simulink library "mec_pointmass_generic_ATvoith_DIWA_NXT"  (R2016a)
settings: Solver=ode45  SolverMode=SingleTasking  StartTime=0.0  StopTime=10.0  RelTol=1e-3
undefined symbols (not defined in the file): sMP
(part 4 of 4)

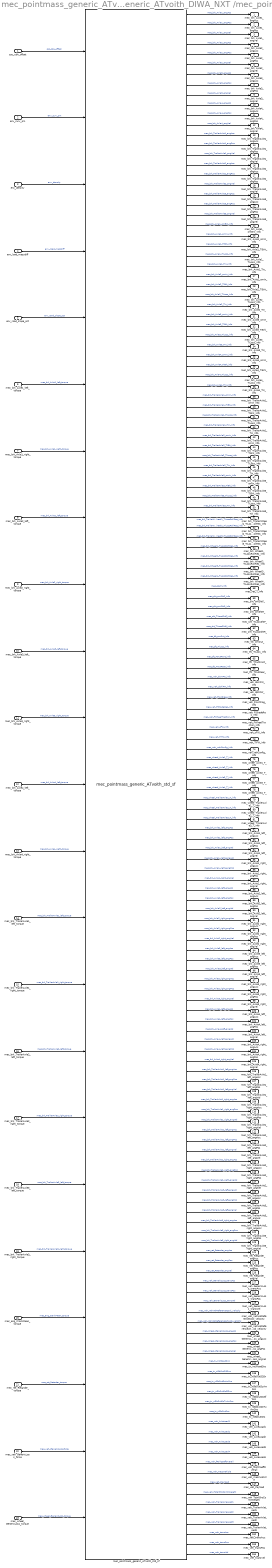
== system mec_pointmass_generic_ATvoith_DIWA_NXT/mec_pointmass_generic_ATvoith_DIWA_NXT /mec_pointmass_generic_ATvoith_std ==
  cpc_cdA_offset : Inport
  env_curv_pm : Inport  Port=2
  env_density : Inport  Port=3
  env_load_massdiff : Inport  Port=4
  env_road_slope_pct : Inport  Port=5
  mec_brk_Axle1_left_torque : Inport  Port=6
  mec_brk_Axle1_right_torque : Inport  Port=7
  mec_brk_Axle2_left_torque : Inport  Port=8
  mec_brk_Axle2_right_torque : Inport  Port=9
  mec_brk_Axle3_left_torque : Inport  Port=10
  mec_brk_Axle3_right_torque : Inport  Port=11
  mec_brk_Axle4_left_torque : Inport  Port=12
  mec_brk_Axle4_right_torque : Inport  Port=13
  mec_brk_TrailerAxle1_left_torque : Inport  Port=14
  mec_brk_TrailerAxle1_right_torque : Inport  Port=15
  mec_brk_TrailerAxle2_left_torque : Inport  Port=16
  mec_brk_TrailerAxle2_right_torque : Inport  Port=17
  mec_brk_TrailerAxle3_left_torque : Inport  Port=18
  mec_brk_TrailerAxle3_right_torque : Inport  Port=19
  mec_eng_CrankMean_torque : Inport  Port=20
  mec_ret_Retarder_torque : Inport  Port=21
  mec_veh_GenericLoss_force : Inport  Port=22
  mec_wheel_GenericLoss_torque : Inport  Port=23
  mec_pointmass_generic_ATvoith_std_sf : S-Function  FunctionName=mec_pointmass_generic_ATvoith_std_sf  Parameters=s1 s2 p1 p2 p3 p4 p5 p6 p7 p8 p9 p10 p11 p12 p13 p14 p15 p16 p17 p18 p19 p20 p21 p22 p23 p24 p25 p26 p27 p28 p29 p30 p31 p32 p33 p34 p35 p36 p37 p38 p39 p40 p41 p42 p43 p44 p45 p46 p47 p48 p49 p50 p51 p52 p53 p54 p55 p56 p57 p58 p59 p60 p61 p62 p63 p64 p65 p66 p67 p68 p69 p70 p71 p72 p73 p74 p75 p76 p77 p78 p79 p80 p81 p82 p83 p84 p85 p86 p87 p88 p89 p90 p91 p92 p93 p94 p95 p96 p97 p98 p99 p100 p101 p102 p103 p104 p105 p106 p107 p108 p109 p110 p111 p112 p113 p114 p115 p116 p117 p118 p119 p120 p121 p122 p123 p124 p125 p126 p127 p128 p129 p130 p131 p132 p133 p134 p135 p136 p137 p138 p139 p140 p141 p142 p143 p144 p145 p146 p147 p148 p149 p150 p151 p152 p153 p154 p155 p156 p157 p158 p159 p160 p161 p162 p163 p164 p165 p166 p167 p168 p169 p170 p171 p172 p173 p174 p175 p176 p177 p178 p179 p180 p181 p182 p183 p184 p185 p186 p187 p188 p189 p190 p191 p192 p193 p194 p195 p196 p197 p198 p199 p200 p201 p202 p203 p204 p205 p206 p207 p208 p209 p210 p211 p212 p213 p214 p215 p216 p217 p218 p219 p220 p221 p222 p223 p224 p225 p226 p227 p228 p229 p230 p231 p232 p233 p234 p235 p236 p237 p238 p239 p240 p241 p242 p243 p244 p245 p246 p247 p248 p249 p250 p251 p252 p253 p254 p255 p256 p257 p258 p259 p260 p261 p262 p263 p264 p265 p266 p267 p268 p269 p270 p271 p272 p273 p274 p275 p276 p277 p278 p279 p280 p281 p282 p283 p284 p285 p286 p287 p288 p289 p290 p291 p292 p293 p294 p295 p296 p297 p298 p299 p300  SFunctionModules=<binary blob, 819 chars, not shown>  SFunctionDeploymentMode=off  EnableBusSupport=off  mask{s1=s1, s2=s2, initCmd='Parameters_mec_pointmass_generic_ATvoith_std_sf', p1=p1, p2=p2, p3=p3, p4=p4, p5=p5, p6=p6, p7=p7, p8=p8, p9=p9, p10=p10, p11=p11, p12=p12, p13=p13, p14=p14, p15=p15, p16=p16, p17=p17, p18=p18, p19=p19, p20=p20, p21=p21, p22=p22, p23=p23, p24=p24, p25=p25, p26=p26, p27=p27, p28=p28, p29=p29, p30=p30, p31=p31, p32=p32, p33=p33, p34=p34, p35=p35, p36=p36, p37=p37, p38=p38, p39=p39, p40=p40, p41=p41, p42=p42, p43=p43, p44=p44, p45=p45, p46=p46, p47=p47, p48=p48, p49=p49, p50=p50, p51=p51, p52=p52, p53=p53, p54=p54, p55=p55, p56=p56, p57=p57, p58=p58, p59=p59, p60=p60, p61=p61, p62=p62, p63=p63, p64=p64, p65=p65, p66=p66, p67=p67, p68=p68, p69=p69, p70=p70, p71=p71, p72=p72, p73=p73, p74=p74, p75=p75, p76=p76, p77=p77, p78=p78, p79=p79, p80=p80, p81=p81, p82=p82, p83=p83, p84=p84, p85=p85, p86=p86, p87=p87, p88=p88, p89=p89, p90=p90, p91=p91, p92=p92, p93=p93, p94=p94, p95=p95, p96=p96, p97=p97, p98=p98, p99=p99, p100=p100, p101=p101, p102=p102, p103=p103, p104=p104, p105=p105, p106=p106, p107=p107, p108=p108, p109=p109, p110=p110, p111=p111, p112=p112, p113=p113, p114=p114, p115=p115, p116=p116, p117=p117, p118=p118, p119=p119, p120=p120, p121=p121, p122=p122, p123=p123, p124=p124, p125=p125, p126=p126, p127=p127, p128=p128, p129=p129, p130=p130, p131=p131, p132=p132, p133=p133, p134=p134, p135=p135, p136=p136, p137=p137, p138=p138, p139=p139, p140=p140, p141=p141, p142=p142, p143=p143, p144=p144, p145=p145, p146=p146, p147=p147, p148=p148, p149=p149, p150=p150, p151=p151, p152=p152, p153=p153, p154=p154, p155=p155, p156=p156, p157=p157, p158=p158, p159=p159, p160=p160, p161=p161, p162=p162, p163=p163, p164=p164, p165=p165, p166=p166, p167=p167, p168=p168, p169=p169, p170=p170, p171=p171, p172=p172, p173=p173, p174=p174, p175=p175, p176=p176, p177=p177, p178=p178, p179=p179, p180=p180, p181=p181, p182=p182, p183=p183, p184=p184, p185=p185, p186=p186, p187=p187, p188=p188, p189=p189, p190=p190, p191=p191, p192=p192, p193=p193, p194=p194, p195=p195, p196=p196, p197=p197, p198=p198, p199=p199, p200=p200, p201=p201, p202=p202, p203=p203, p204=p204, p205=p205, p206=p206, p207=p207, p208=p208, p209=p209, p210=p210, p211=p211, p212=p212, p213=p213, p214=p214, p215=p215, p216=p216, p217=p217, p218=p218, p219=p219, p220=p220, p221=p221, p222=p222, p223=p223, p224=p224, p225=p225, p226=p226, p227=p227, p228=p228, p229=p229, p230=p230, p231=p231, p232=p232, p233=p233, p234=p234, p235=p235, p236=p236, p237=p237, p238=p238, p239=p239, p240=p240, p241=p241, p242=p242, p243=p243, p244=p244, p245=p245, p246=p246, p247=p247, p248=p248, p249=p249, p250=p250, p251=p251, p252=p252, p253=p253, p254=p254, p255=p255, p256=p256, p257=p257, p258=p258, p259=p259, p260=p260, p261=p261, p262=p262, p263=p263, p264=p264, p265=p265, p266=p266, p267=p267, p268=p268, p269=p269, p270=p270, p271=p271, p272=p272, p273=p273, p274=p274, p275=p275, p276=p276, p277=p277, p278=p278, p279=p279, p280=p280, p281=p281, p282=p282, p283=p283, p284=p284, p285=p285, p286=p286, p287=p287, p288=p288, p289=p289, p290=p290, p291=p291, p292=p292, p293=p293, p294=p294, p295=p295, p296=p296, p297=p297, p298=p298, p299=p299, p300=p300}
      mask prompts: s1 "Solver Type: settings_iMode [-]"; s2 "Solver Step Size: settings_dt [s]"; initCmd "Initialization command"; p1 "Ratio Differential Gear [-] export=true name=iDiff prio=1 dataSetName=axle_dummy dataClassType=axle dataClassName=$dataClassNameAxle$ moduleXmlReference=$moduleXmlReferenceAxle$ unit='-' description='Ratio Differential Gear': axle1.iDiff [-]"; p2 "Is driven Axle? [-] export=true name=isDriven prio=1 dataSetName=axle_dummy dataClassType=axle dataClassName=$dataClassNameAxle$ moduleXmlReference=$moduleXmlReferenceAxle$ unit='-' description='Is Driven Axle': axle1.isDriven [-]"; p3 "Is rear Axle? [-] export=true name=isRearAxle prio=1 dataSetName=axle_dummy dataClassType=axle dataClassName=$dataClassNameAxle$ moduleXmlReference=$moduleXmlReferenceAxle$ unit='-' description='Is Rear Axle': axle1.isRearAxle [-]"; p4 "Inertia Brake Disc  [kgm^2] export=true name=JBrakeDisc_kgm2 prio=1 dataSetName=brk_dummy dataClassType=brk dataClassName=$dataClassNameBrk$ moduleXmlReference=$moduleXmlReferenceBrk$ unit='kgm^2' description='Inertia Brake Disc': axle1.JBrakeDisc_kgm2 [kgm²]"; p5 "Inertia Hub  [kgm^2] export=true name=JHub_kgm2 prio=1 dataSetName=brk_dummy dataClassType=brk dataClassName=$dataClassNameBrk$ moduleXmlReference=$moduleXmlReferenceBrk$ unit='kgm^2' description='Inertia Hub': axle1.JHub_kgm2 [-]"; p6 "Inertia Side Shaft [kgm^2] export=true name=JSideShft_kgm2 prio=1 dataSetName=axle_dummy dataClassType=axle dataClassName=$dataClassNameAxle$ moduleXmlReference=$moduleXmlReferenceAxle$ unit='kgm^2' description='Inertia Side Shaft': axle1.JSideShft_kgm2 [kgm²]"; p7 "Ratio Differential Gear [-] export=true name=iDiff prio=1 dataSetName=axle_dummy dataClassType=axle dataClassName=$dataClassNameAxle$ moduleXmlReference=$moduleXmlReferenceAxle$ unit='-' description='Ratio Differential Gear': axle2.iDiff [-]"; p8 "Is driven Axle? [-] export=true name=isDriven prio=1 dataSetName=axle_dummy dataClassType=axle dataClassName=$dataClassNameAxle$ moduleXmlReference=$moduleXmlReferenceAxle$ unit='-' description='Is Driven Axle': axle2.isDriven [-]"; p9 "Is rear Axle? [-] export=true name=isRearAxle prio=1 dataSetName=axle_dummy dataClassType=axle dataClassName=$dataClassNameAxle$ moduleXmlReference=$moduleXmlReferenceAxle$ unit='-' description='Is Rear Axle': axle2.isRearAxle [-]"; p10 "Inertia Brake Disc  [kgm^2] export=true name=JBrakeDisc_kgm2 prio=1 dataSetName=brk_dummy dataClassType=brk dataClassName=$dataClassNameBrk$ moduleXmlReference=$moduleXmlReferenceBrk$ unit='kgm^2' description='Inertia Brake Disc': axle2.JBrakeDisc_kgm2 [kgm²]"; p11 "Inertia Hub  [kgm^2] export=true name=JHub_kgm2 prio=1 dataSetName=brk_dummy dataClassType=brk dataClassName=$dataClassNameBrk$ moduleXmlReference=$moduleXmlReferenceBrk$ unit='kgm^2' description='Inertia Hub': axle2.JHub_kgm2 [-]"; p12 "Inertia Side Shaft [kgm^2] export=true name=JSideShft_kgm2 prio=1 dataSetName=axle_dummy dataClassType=axle dataClassName=$dataClassNameAxle$ moduleXmlReference=$moduleXmlReferenceAxle$ unit='kgm^2' description='Inertia Side Shaft': axle2.JSideShft_kgm2 [kgm²]"; p13 "Ratio Differential Gear [-] export=true name=iDiff prio=1 dataSetName=axle_dummy dataClassType=axle dataClassName=$dataClassNameAxle$ moduleXmlReference=$moduleXmlReferenceAxle$ unit='-' description='Ratio Differential Gear': axle3.iDiff [-]"; p14 "Is driven Axle? [-] export=true name=isDriven prio=1 dataSetName=axle_dummy dataClassType=axle dataClassName=$dataClassNameAxle$ moduleXmlReference=$moduleXmlReferenceAxle$ unit='-' description='Is Driven Axle': axle3.isDriven [-]"; p15 "Is rear Axle? [-] export=true name=isRearAxle prio=1 dataSetName=axle_dummy dataClassType=axle dataClassName=$dataClassNameAxle$ moduleXmlReference=$moduleXmlReferenceAxle$ unit='-' description='Is Rear Axle': axle3.isRearAxle [-]"; p16 "Inertia Brake Disc  [kgm^2] export=true name=JBrakeDisc_kgm2 prio=1 dataSetName=brk_dummy dataClassType=brk dataClassName=$dataClassNameBrk$ moduleXmlReference=$moduleXmlReferenceBrk$ unit='kgm^2' description='Inertia Brake Disc': axle3.JBrakeDisc_kgm2 [kgm²]"; p17 "Inertia Hub  [kgm^2] export=true name=JHub_kgm2 prio=1 dataSetName=brk_dummy dataClassType=brk dataClassName=$dataClassNameBrk$ moduleXmlReference=$moduleXmlReferenceBrk$ unit='kgm^2' description='Inertia Hub': axle3.JHub_kgm2 [-]"; p18 "Inertia Side Shaft [kgm^2] export=true name=JSideShft_kgm2 prio=1 dataSetName=axle_dummy dataClassType=axle dataClassName=$dataClassNameAxle$ moduleXmlReference=$moduleXmlReferenceAxle$ unit='kgm^2' description='Inertia Side Shaft': axle3.JSideShft_kgm2 [kgm²]"; p19 "Ratio Differential Gear [-] export=true name=iDiff prio=1 dataSetName=axle_dummy dataClassType=axle dataClassName=$dataClassNameAxle$ moduleXmlReference=$moduleXmlReferenceAxle$ unit='-' description='Ratio Differential Gear': axle4.iDiff [-]"; p20 "Is driven Axle? [-] export=true name=isDriven prio=1 dataSetName=axle_dummy dataClassType=axle dataClassName=$dataClassNameAxle$ moduleXmlReference=$moduleXmlReferenceAxle$ unit='-' description='Is Driven Axle': axle4.isDriven [-]"; p21 "Is rear Axle? [-] export=true name=isRearAxle prio=1 dataSetName=axle_dummy dataClassType=axle dataClassName=$dataClassNameAxle$ moduleXmlReference=$moduleXmlReferenceAxle$ unit='-' description='Is Rear Axle': axle4.isRearAxle [-]"; p22 "Inertia Brake Disc  [kgm^2] export=true name=JBrakeDisc_kgm2 prio=1 dataSetName=brk_dummy dataClassType=brk dataClassName=$dataClassNameBrk$ moduleXmlReference=$moduleXmlReferenceBrk$ unit='kgm^2' description='Inertia Brake Disc': axle4.JBrakeDisc_kgm2 [kgm²]"; p23 "Inertia Hub  [kgm^2] export=true name=JHub_kgm2 prio=1 dataSetName=brk_dummy dataClassType=brk dataClassName=$dataClassNameBrk$ moduleXmlReference=$moduleXmlReferenceBrk$ unit='kgm^2' description='Inertia Hub': axle4.JHub_kgm2 [-]"; p24 "Inertia Side Shaft [kgm^2] export=true name=JSideShft_kgm2 prio=1 dataSetName=axle_dummy dataClassType=axle dataClassName=$dataClassNameAxle$ moduleXmlReference=$moduleXmlReferenceAxle$ unit='kgm^2' description='Inertia Side Shaft': axle4.JSideShft_kgm2 [kgm²]"; p25 "Additive Controlable Air Resistance (init) export=$sw_cpc_cdA_offset$ name=cpc_cdA_offset prio=1 dataSetName=std dataClassType=initIO dataClassName=initIO unit='' description='Additive Controlable Air Resistance': interface_IO.cpc_cdA_offset_0 [-]"; p26 "Curve Curvature (init) export=$sw_env_curv_pm$ name=env_curv_pm prio=1 dataSetName=std dataClassType=initIO dataClassName=initIO unit='1/m' description='Curve Curvature': interface_IO.env_curv_pm_0 [-]"; p27 "Air density from environment (init) export=$sw_env_density$ name=env_density prio=1 dataSetName=std dataClassType=initIO dataClassName=initIO unit='kg/m^3' description='Air density from environment': interface_IO.env_density_0 [-]"; p28 "Mass Difference (init) export=$sw_env_load_massdiff$ name=env_load_massdiff prio=1 dataSetName=std dataClassType=initIO dataClassName=initIO unit='1/m' description='Curve Curvature': interface_IO.env_load_massdiff_0 [-]"; p29 "Slope of road from environment (init) export=$sw_env_road_slope_pct$ name=env_road_slope_pct prio=1 dataSetName=std dataClassType=initIO dataClassName=initIO unit='-' description='Slope of road from environment': interface_IO.env_road_slope_pct_0 [-]"; p30 "Acceleration Brake 1 (init) export=$sw_mec_brk_Axle1_angAcc$ name=mec_brk_Axle1_angAcc prio=1 dataSetName=std dataClassType=initIO dataClassName=initIO unit='rad/s^2' description='Acceleration Brake 1': interface_IO.mec_brk_Axle1_angAcc_0 [-]"; p31 "Angle Brake 1 (init) export=$sw_mec_brk_Axle1_angPos$ name=mec_brk_Axle1_angPos prio=1 dataSetName=std dataClassType=initIO dataClassName=initIO unit='rad' description='Angle Brake 1': interface_IO.mec_brk_Axle1_angPos_0 [-]"; p32 "Velocity Brake 1 (init) export=$sw_mec_brk_Axle1_angVel$ name=mec_brk_Axle1_angVel prio=1 dataSetName=std dataClassType=initIO dataClassName=initIO unit='rad/s' description='Velocity Brake 1': interface_IO.mec_brk_Axle1_angVel_0 [-]"; p33 "Acceleration Brake 1 left Wheel (init) export=$sw_mec_brk_Axle1_left_angAcc$ name=mec_brk_Axle1_left_angAcc prio=1 dataSetName=std dataClassType=initIO dataClassName=initIO unit='rad/s^2' description='Acceleration Brake 1 left Wheel': interface_IO.mec_brk_Axle1_left_angAcc_0 [-]"; p34 "Angle Brake 1 left Wheel (init) export=$sw_mec_brk_Axle1_left_angPos$ name=mec_brk_Axle1_left_angPos prio=1 dataSetName=std dataClassType=initIO dataClassName=initIO unit='rad' description='Angle Brake 1 left Wheel': interface_IO.mec_brk_Axle1_left_angPos_0 [-]"; p35 "Velocity Brake 1 left Wheel (init) export=$sw_mec_brk_Axle1_left_angVel$ name=mec_brk_Axle1_left_angVel prio=1 dataSetName=std dataClassType=initIO dataClassName=initIO unit='rad/s' description='Velocity Brake 1 left Wheel': interface_IO.mec_brk_Axle1_left_angVel_0 [-]"; p36 "Torque Brake 1 left Wheel (init) export=$sw_mec_brk_Axle1_left_torque$ name=mec_brk_Axle1_left_torque prio=1 dataSetName=std dataClassType=initIO dataClassName=initIO unit='Nm' description='Torque Brake 1 left Wheel': interface_IO.mec_brk_Axle1_left_torque_0 [-]"; p37 "Acceleration Brake 1 right Wheel (init) export=$sw_mec_brk_Axle1_right_angAcc$ name=mec_brk_Axle1_right_angAcc prio=1 dataSetName=std dataClassType=initIO dataClassName=initIO unit='rad/s^2' description='Acceleration Brake 1 right Wheel': interface_IO.mec_brk_Axle1_right_angAcc_0 [-]"; p38 "Angle Brake 1 right Wheel (init) export=$sw_mec_brk_Axle1_right_angPos$ name=mec_brk_Axle1_right_angPos prio=1 dataSetName=std dataClassType=initIO dataClassName=initIO unit='rad' description='Angle Brake 1 right Wheel': interface_IO.mec_brk_Axle1_right_angPos_0 [-]"; p39 "Velocity Brake 1 right Wheel (init) export=$sw_mec_brk_Axle1_right_angVel$ name=mec_brk_Axle1_right_angVel prio=1 dataSetName=std dataClassType=initIO dataClassName=initIO unit='rad/s' description='Velocity Brake 1 right Wheel': interface_IO.mec_brk_Axle1_right_angVel_0 [-]"; p40 "Torque Brake 1 left Wheel (init) export=$sw_mec_brk_Axle1_right_torque$ name=mec_brk_Axle1_right_torque prio=1 dataSetName=std dataClassType=initIO dataClassName=initIO unit='Nm' description='Torque Brake 1 left Wheel': interface_IO.mec_brk_Axle1_right_torque_0 [-]"; p41 "Acceleration Brake 2 (init) export=$sw_mec_brk_Axle2_angAcc$ name=mec_brk_Axle2_angAcc prio=1 dataSetName=std dataClassType=initIO dataClassName=initIO unit='rad/s^2' description='Acceleration Brake 2': interface_IO.mec_brk_Axle2_angAcc_0 [-]"; p42 "Angle Brake 2 (init) export=$sw_mec_brk_Axle2_angPos$ name=mec_brk_Axle2_angPos prio=1 dataSetName=std dataClassType=initIO dataClassName=initIO unit='rad' description='Angle Brake 2': interface_IO.mec_brk_Axle2_angPos_0 [-]"; p43 "Velocity Brake 2 (init) export=$sw_mec_brk_Axle2_angVel$ name=mec_brk_Axle2_angVel prio=1 dataSetName=std dataClassType=initIO dataClassName=initIO unit='rad/s' description='Velocity Brake 3': interface_IO.mec_brk_Axle2_angVel_0 [-]"; p44 "Acceleration Brake 2 left Wheel (init) export=$sw_mec_brk_Axle2_left_angAcc$ name=mec_brk_Axle2_left_angAcc prio=1 dataSetName=std dataClassType=initIO dataClassName=initIO unit='rad/s^2' description='Acceleration Brake 2 left Wheel': interface_IO.mec_brk_Axle2_left_angAcc_0 [-]"; p45 "Angle Brake 2 left Wheel (init) export=$sw_mec_brk_Axle2_left_angPos$ name=mec_brk_Axle2_left_angPos prio=1 dataSetName=std dataClassType=initIO dataClassName=initIO unit='rad' description='Angle Brake 2 left Wheel': interface_IO.mec_brk_Axle2_left_angPos_0 [-]"; p46 "Velocity Brake 2 left Wheel (init) export=$sw_mec_brk_Axle2_left_angVel$ name=mec_brk_Axle2_left_angVel prio=1 dataSetName=std dataClassType=initIO dataClassName=initIO unit='rad/s' description='Velocity Brake 3 left Wheel': interface_IO.mec_brk_Axle2_left_angVel_0 [-]"; p47 "Torque Brake 2 left Wheel (init) export=$sw_mec_brk_Axle2_left_torque$ name=mec_brk_Axle2_left_torque prio=1 dataSetName=std dataClassType=initIO dataClassName=initIO unit='Nm' description='Torque Brake 2 left Wheel': interface_IO.mec_brk_Axle2_left_torque_0 [-]"; p48 "Acceleration Brake 2 right Wheel (init) export=$sw_mec_brk_Axle2_right_angAcc$ name=mec_brk_Axle2_right_angAcc prio=1 dataSetName=std dataClassType=initIO dataClassName=initIO unit='rad/s^2' description='Acceleration Brake 2 right Wheel': interface_IO.mec_brk_Axle2_right_angAcc_0 [-]"; p49 "Angle Brake 2 right Wheel (init) export=$sw_mec_brk_Axle2_right_angPos$ name=mec_brk_Axle2_right_angPos prio=1 dataSetName=std dataClassType=initIO dataClassName=initIO unit='rad' description='Angle Brake 2 right Wheel': interface_IO.mec_brk_Axle2_right_angPos_0 [-]"; p50 "Velocity Brake 2 right Wheel (init) export=$sw_mec_brk_Axle2_right_angVel$ name=mec_brk_Axle2_right_angVel prio=1 dataSetName=std dataClassType=initIO dataClassName=initIO unit='rad/s' description='Velocity Brake 3 right Wheel': interface_IO.mec_brk_Axle2_right_angVel_0 [-]"; p51 "Torque Brake 2 right Wheel (init) export=$sw_mec_brk_Axle2_right_torque$ name=mec_brk_Axle2_right_torque prio=1 dataSetName=std dataClassType=initIO dataClassName=initIO unit='Nm' description='Torque Brake 2 right Wheel': interface_IO.mec_brk_Axle2_right_torque_0 [-]"; p52 "Acceleration Brake 3 (init) export=$sw_mec_brk_Axle3_angAcc$ name=mec_brk_Axle3_angAcc prio=1 dataSetName=std dataClassType=initIO dataClassName=initIO unit='rad/s^2' description='Acceleration Brake 3': interface_IO.mec_brk_Axle3_angAcc_0 [-]"; p53 "Angle Brake 3 (init) export=$sw_mec_brk_Axle3_angPos$ name=mec_brk_Axle3_angPos prio=1 dataSetName=std dataClassType=initIO dataClassName=initIO unit='rad' description='Angle Brake 3': interface_IO.mec_brk_Axle3_angPos_0 [-]"; p54 "Velocity Brake 3 (init) export=$sw_mec_brk_Axle3_angVel$ name=mec_brk_Axle3_angVel prio=1 dataSetName=std dataClassType=initIO dataClassName=initIO unit='rad/s' description='Velocity Brake 3': interface_IO.mec_brk_Axle3_angVel_0 [-]"; p55 "Acceleration Brake 3 left Wheel (init) export=$sw_mec_brk_Axle3_left_angAcc$ name=mec_brk_Axle3_left_angAcc prio=1 dataSetName=std dataClassType=initIO dataClassName=initIO unit='rad/s^2' description='Acceleration Brake 3 left Wheel': interface_IO.mec_brk_Axle3_left_angAcc_0 [-]"; p56 "Angle Brake 3 left Wheel (init) export=$sw_mec_brk_Axle3_left_angPos$ name=mec_brk_Axle3_left_angPos prio=1 dataSetName=std dataClassType=initIO dataClassName=initIO unit='rad' description='Angle Brake 3 left Wheel': interface_IO.mec_brk_Axle3_left_angPos_0 [-]"; p57 "Velocity Brake 3 left Wheel (init) export=$sw_mec_brk_Axle3_left_angVel$ name=mec_brk_Axle3_left_angVel prio=1 dataSetName=std dataClassType=initIO dataClassName=initIO unit='rad/s' description='Velocity Brake 3 left Wheel': interface_IO.mec_brk_Axle3_left_angVel_0 [-]"; p58 "Torque Brake 3 left Wheel (init) export=$sw_mec_brk_Axle3_left_torque$ name=mec_brk_Axle3_left_torque prio=1 dataSetName=std dataClassType=initIO dataClassName=initIO unit='Nm' description='Torque Brake 3 left Wheel': interface_IO.mec_brk_Axle3_left_torque_0 [-]"; p59 "Acceleration Brake 3 right Wheel (init) export=$sw_mec_brk_Axle3_right_angAcc$ name=mec_brk_Axle3_right_angAcc prio=1 dataSetName=std dataClassType=initIO dataClassName=initIO unit='rad/s^2' description='Acceleration Brake 3 right Wheel': interface_IO.mec_brk_Axle3_right_angAcc_0 [-]"; p60 "Angle Brake 3 right Wheel (init) export=$sw_mec_brk_Axle3_right_angPos$ name=mec_brk_Axle3_right_angPos prio=1 dataSetName=std dataClassType=initIO dataClassName=initIO unit='rad' description='Angle Brake 3 right Wheel': interface_IO.mec_brk_Axle3_right_angPos_0 [-]"; p61 "Velocity Brake 3 right Wheel (init) export=$sw_mec_brk_Axle3_right_angVel$ name=mec_brk_Axle3_right_angVel prio=1 dataSetName=std dataClassType=initIO dataClassName=initIO unit='rad/s' description='Velocity Brake 3 right Wheel': interface_IO.mec_brk_Axle3_right_angVel_0 [-]"; p62 "Torque Brake 3 right Wheel (init) export=$sw_mec_brk_Axle3_right_torque$ name=mec_brk_Axle3_right_torque prio=1 dataSetName=std dataClassType=initIO dataClassName=initIO unit='Nm' description='Torque Brake 3 right Wheel': interface_IO.mec_brk_Axle3_right_torque_0 [-]"; p63 "Acceleration Brake 4 (init) export=$sw_mec_brk_Axle4_angAcc$ name=mec_brk_Axle4_angAcc prio=1 dataSetName=std dataClassType=initIO dataClassName=initIO unit='rad/s^2' description='Acceleration Brake 4': interface_IO.mec_brk_Axle4_angAcc_0 [-]"; p64 "Angle Brake 4 (init) export=$sw_mec_brk_Axle4_angPos$ name=mec_brk_Axle4_angPos prio=1 dataSetName=std dataClassType=initIO dataClassName=initIO unit='rad' description='Angle Brake 4': interface_IO.mec_brk_Axle4_angPos_0 [-]"; p65 "Velocity Brake 4 (init) export=$sw_mec_brk_Axle4_angVel$ name=mec_brk_Axle4_angVel prio=1 dataSetName=std dataClassType=initIO dataClassName=initIO unit='rad/s' description='Velocity Brake 4': interface_IO.mec_brk_Axle4_angVel_0 [-]"; p66 "Acceleration Brake 4 left Wheel (init) export=$sw_mec_brk_Axle4_left_angAcc$ name=mec_brk_Axle4_left_angAcc prio=1 dataSetName=std dataClassType=initIO dataClassName=initIO unit='rad/s^2' description='Acceleration Brake 4 left Wheel': interface_IO.mec_brk_Axle4_left_angAcc_0 [-]"; p67 "Angle Brake 4 left Wheel (init) export=$sw_mec_brk_Axle4_left_angPos$ name=mec_brk_Axle4_left_angPos prio=1 dataSetName=std dataClassType=initIO dataClassName=initIO unit='rad' description='Angle Brake 4 left Wheel': interface_IO.mec_brk_Axle4_left_angPos_0 [-]"; p68 "Velocity Brake 4 left Wheel (init) export=$sw_mec_brk_Axle4_left_angVel$ name=mec_brk_Axle4_left_angVel prio=1 dataSetName=std dataClassType=initIO dataClassName=initIO unit='rad/s' description='Velocity Brake 4 left Wheel': interface_IO.mec_brk_Axle4_left_angVel_0 [-]"; p69 "Torque Brake 4 left Wheel (init) export=$sw_mec_brk_Axle4_left_torque$ name=mec_brk_Axle4_left_torque prio=1 dataSetName=std dataClassType=initIO dataClassName=initIO unit='Nm' description='Torque Brake 4 left Wheel': interface_IO.mec_brk_Axle4_left_torque_0 [-]"; p70 "Acceleration Brake 4 right Wheel (init) export=$sw_mec_brk_Axle4_right_angAcc$ name=mec_brk_Axle4_right_angAcc prio=1 dataSetName=std dataClassType=initIO dataClassName=initIO unit='rad/s^2' description='Acceleration Brake 4 right Wheel': interface_IO.mec_brk_Axle4_right_angAcc_0 [-]"; p71 "Angle Brake 4 right Wheel (init) export=$sw_mec_brk_Axle4_right_angPos$ name=mec_brk_Axle4_right_angPos prio=1 dataSetName=std dataClassType=initIO dataClassName=initIO unit='rad' description='Angle Brake 4 right Wheel': interface_IO.mec_brk_Axle4_right_angPos_0 [-]"; p72 "Velocity Brake 4 right Wheel (init) export=$sw_mec_brk_Axle4_right_angVel$ name=mec_brk_Axle4_right_angVel prio=1 dataSetName=std dataClassType=initIO dataClassName=initIO unit='rad/s' description='Velocity Brake 4 right Wheel': interface_IO.mec_brk_Axle4_right_angVel_0 [-]"; p73 "Torque Brake 4 right Wheel (init) export=$sw_mec_brk_Axle4_right_torque$ name=mec_brk_Axle4_right_torque prio=1 dataSetName=std dataClassType=initIO dataClassName=initIO unit='Nm' description='Torque Brake 4 right Wheel': interface_IO.mec_brk_Axle4_right_torque_0 [-]"; p74 "Acceleration Trailer Brake 1 (init) export=$sw_mec_brk_TrailerAxle1_angAcc$ name=mec_brk_TrailerAxle1_angAcc prio=1 dataSetName=std dataClassType=initIO dataClassName=initIO unit='rad/s^2' description='Acceleration Trailer Brake 1': interface_IO.mec_brk_TrailerAxle1_angAcc_0 [-]"; p75 "Angle Trailer Brake 1 (init) export=$sw_mec_brk_TrailerAxle1_angPos$ name=mec_brk_TrailerAxle1_angPos prio=1 dataSetName=std dataClassType=initIO dataClassName=initIO unit='rad' description='Angle Trailer Brake 1': interface_IO.mec_brk_TrailerAxle1_angPos_0 [-]"; p76 "Velocity Trailer Brake 1 (init) export=$sw_mec_brk_TrailerAxle1_angVel$ name=mec_brk_TrailerAxle1_angVel prio=1 dataSetName=std dataClassType=initIO dataClassName=initIO unit='rad/s' description='Velocity Trailer Brake 1': interface_IO.mec_brk_TrailerAxle1_angVel_0 [-]"; p77 "Acceleration Trailer Brake 1 left Wheel (init) export=$sw_mec_brk_TrailerAxle1_left_angAcc$ name=mec_brk_TrailerAxle1_left_angAcc prio=1 dataSetName=std dataClassType=initIO dataClassName=initIO unit='rad/s^2' description='Acceleration Trailer Brake 1 left Wheel': interface_IO.mec_brk_TrailerAxle1_left_angAcc_0 [-]"; p78 "Angle Trailer Brake 1 left Wheel (init) export=$sw_mec_brk_TrailerAxle1_left_angPos$ name=mec_brk_TrailerAxle1_left_angPos prio=1 dataSetName=std dataClassType=initIO dataClassName=initIO unit='rad' description='Angle Trailer Brake 1 left Wheel': interface_IO.mec_brk_TrailerAxle1_left_angPos_0 [-]"; p79 "Velocity Trailer Brake 1 left Wheel (init) export=$sw_mec_brk_TrailerAxle1_left_angVel$ name=mec_brk_TrailerAxle1_left_angVel prio=1 dataSetName=std dataClassType=initIO dataClassName=initIO unit='rad/s' description='Velocity Trailer Brake 1 left Wheel': interface_IO.mec_brk_TrailerAxle1_left_angVel_0 [-]"; p80 "Torque Trailer Brake 1 left Wheel (init) export=$sw_mec_brk_TrailerAxle1_left_torque$ name=mec_brk_TrailerAxle1_left_torque prio=1 dataSetName=std dataClassType=initIO dataClassName=initIO unit='Nm' description='Torque Trailer Brake 1 left Wheel': interface_IO.mec_brk_TrailerAxle1_left_torque_0 [-]"; p81 "Acceleration Trailer Brake 1 right Wheel (init) export=$sw_mec_brk_TrailerAxle1_right_angAcc$ name=mec_brk_TrailerAxle1_right_angAcc prio=1 dataSetName=std dataClassType=initIO dataClassName=initIO unit='rad/s^2' description='Acceleration Trailer Brake 1 right Wheel': interface_IO.mec_brk_TrailerAxle1_right_angAcc_0 [-]"; p82 "Angle Trailer Brake 1 right Wheel (init) export=$sw_mec_brk_TrailerAxle1_right_angPos$ name=mec_brk_TrailerAxle1_right_angPos prio=1 dataSetName=std dataClassType=initIO dataClassName=initIO unit='rad' description='Angle Trailer Brake 1 right Wheel': interface_IO.mec_brk_TrailerAxle1_right_angPos_0 [-]"; p83 "Velocity Trailer Brake 1 right Wheel (init) export=$sw_mec_brk_TrailerAxle1_right_angVel$ name=mec_brk_TrailerAxle1_right_angVel prio=1 dataSetName=std dataClassType=initIO dataClassName=initIO unit='rad/s' description='Velocity Trailer Brake 1 right Wheel': interface_IO.mec_brk_TrailerAxle1_right_angVel_0 [-]"; p84 "Torque Trailer Brake 1 right Wheel (init) export=$sw_mec_brk_TrailerAxle1_right_torque$ name=mec_brk_TrailerAxle1_right_torque prio=1 dataSetName=std dataClassType=initIO dataClassName=initIO unit='Nm' description='Torque Trailer Brake 1 right Wheel': interface_IO.mec_brk_TrailerAxle1_right_torque_0 [-]"; p85 "Acceleration Trailer Brake 2 (init) export=$sw_mec_brk_TrailerAxle2_angAcc$ name=mec_brk_TrailerAxle2_angAcc prio=1 dataSetName=std dataClassType=initIO dataClassName=initIO unit='rad/s^2' description='Acceleration Trailer Brake 2': interface_IO.mec_brk_TrailerAxle2_angAcc_0 [-]"; p86 "Angle Trailer Brake 2 (init) export=$sw_mec_brk_TrailerAxle2_angPos$ name=mec_brk_TrailerAxle2_angPos prio=1 dataSetName=std dataClassType=initIO dataClassName=initIO unit='rad' description='Angle Trailer Brake 2': interface_IO.mec_brk_TrailerAxle2_angPos_0 [-]"; p87 "Velocity Trailer Brake 2 (init) export=$sw_mec_brk_TrailerAxle2_angVel$ name=mec_brk_TrailerAxle2_angVel prio=1 dataSetName=std dataClassType=initIO dataClassName=initIO unit='rad/s' description='Velocity Trailer Brake 2': interface_IO.mec_brk_TrailerAxle2_angVel_0 [-]"; p88 "Acceleration Trailer Brake 2 left Wheel (init) export=$sw_mec_brk_TrailerAxle2_left_angAcc$ name=mec_brk_TrailerAxle2_left_angAcc prio=1 dataSetName=std dataClassType=initIO dataClassName=initIO unit='rad/s^2' description='Acceleration Trailer Brake 2 left Wheel': interface_IO.mec_brk_TrailerAxle2_left_angAcc_0 [-]"; p89 "Angle Trailer Brake 2 left Wheel (init) export=$sw_mec_brk_TrailerAxle2_left_angPos$ name=mec_brk_TrailerAxle2_left_angPos prio=1 dataSetName=std dataClassType=initIO dataClassName=initIO unit='rad' description='Angle Trailer Brake 2 left Wheel': interface_IO.mec_brk_TrailerAxle2_left_angPos_0 [-]"; p90 "Velocity Trailer Brake 2 left Wheel (init) export=$sw_mec_brk_TrailerAxle2_left_angVel$ name=mec_brk_TrailerAxle2_left_angVel prio=1 dataSetName=std dataClassType=initIO dataClassName=initIO unit='rad/s' description='Velocity Trailer Brake 2 left Wheel': interface_IO.mec_brk_TrailerAxle2_left_angVel_0 [-]"; p91 "Torque Trailer Brake 2 left Wheel (init) export=$sw_mec_brk_TrailerAxle2_left_torque$ name=mec_brk_TrailerAxle2_left_torque prio=1 dataSetName=std dataClassType=initIO dataClassName=initIO unit='Nm' description='Torque Trailer Brake 2 left Wheel': interface_IO.mec_brk_TrailerAxle2_left_torque_0 [-]"; p92 "Acceleration Trailer Brake 2 right Wheel (init) export=$sw_mec_brk_TrailerAxle2_right_angAcc$ name=mec_brk_TrailerAxle2_right_angAcc prio=1 dataSetName=std dataClassType=initIO dataClassName=initIO unit='rad/s^2' description='Acceleration Trailer Brake 2 right Wheel': interface_IO.mec_brk_TrailerAxle2_right_angAcc_0 [-]"; p93 "Angle Trailer Brake 2 right Wheel (init) export=$sw_mec_brk_TrailerAxle2_right_angPos$ name=mec_brk_TrailerAxle2_right_angPos prio=1 dataSetName=std dataClassType=initIO dataClassName=initIO unit='rad' description='Angle Trailer Brake 2 right Wheel': interface_IO.mec_brk_TrailerAxle2_right_angPos_0 [-]"; p94 "Velocity Trailer Brake 2 right Wheel (init) export=$sw_mec_brk_TrailerAxle2_right_angVel$ name=mec_brk_TrailerAxle2_right_angVel prio=1 dataSetName=std dataClassType=initIO dataClassName=initIO unit='rad/s' description='Velocity Trailer Brake 2 right Wheel': interface_IO.mec_brk_TrailerAxle2_right_angVel_0 [-]"; p95 "Torque Trailer Brake 2 right Wheel (init) export=$sw_mec_brk_TrailerAxle2_right_torque$ name=mec_brk_TrailerAxle2_right_torque prio=1 dataSetName=std dataClassType=initIO dataClassName=initIO unit='Nm' description='Torque Trailer Brake 2 right Wheel': interface_IO.mec_brk_TrailerAxle2_right_torque_0 [-]"; p96 "Acceleration Trailer Brake 3 (init) export=$sw_mec_brk_TrailerAxle3_angAcc$ name=mec_brk_TrailerAxle3_angAcc prio=1 dataSetName=std dataClassType=initIO dataClassName=initIO unit='rad/s^2' description='Acceleration Trailer Brake 3': interface_IO.mec_brk_TrailerAxle3_angAcc_0 [-]"; p97 "Angle Trailer Brake 3 (init) export=$sw_mec_brk_TrailerAxle3_angPos$ name=mec_brk_TrailerAxle3_angPos prio=1 dataSetName=std dataClassType=initIO dataClassName=initIO unit='rad' description='Angle Trailer Brake 3': interface_IO.mec_brk_TrailerAxle3_angPos_0 [-]"; p98 "Velocity Trailer Brake 3 (init) export=$sw_mec_brk_TrailerAxle3_angVel$ name=mec_brk_TrailerAxle3_angVel prio=1 dataSetName=std dataClassType=initIO dataClassName=initIO unit='rad/s' description='Velocity Trailer Brake 3': interface_IO.mec_brk_TrailerAxle3_angVel_0 [-]"; p99 "Acceleration Trailer Brake 3 left Wheel (init) export=$sw_mec_brk_TrailerAxle3_left_angAcc$ name=mec_brk_TrailerAxle3_left_angAcc prio=1 dataSetName=std dataClassType=initIO dataClassName=initIO unit='rad/s^2' description='Acceleration Trailer Brake 3 left Wheel': interface_IO.mec_brk_TrailerAxle3_left_angAcc_0 [-]"; p100 "Angle Trailer Brake 3 left Wheel (init) export=$sw_mec_brk_TrailerAxle3_left_angPos$ name=mec_brk_TrailerAxle3_left_angPos prio=1 dataSetName=std dataClassType=initIO dataClassName=initIO unit='rad' description='Angle Trailer Brake 3 left Wheel': interface_IO.mec_brk_TrailerAxle3_left_angPos_0 [-]"; p101 "Velocity Trailer Brake 3 left Wheel (init) export=$sw_mec_brk_TrailerAxle3_left_angVel$ name=mec_brk_TrailerAxle3_left_angVel prio=1 dataSetName=std dataClassType=initIO dataClassName=initIO unit='rad/s' description='Velocity Trailer Brake 3 left Wheel': interface_IO.mec_brk_TrailerAxle3_left_angVel_0 [-]"; p102 "Torque Trailer Brake 3 left Wheel (init) export=$sw_mec_brk_TrailerAxle3_left_torque$ name=mec_brk_TrailerAxle3_left_torque prio=1 dataSetName=std dataClassType=initIO dataClassName=initIO unit='Nm' description='Torque Trailer Brake 3  left Wheel': interface_IO.mec_brk_TrailerAxle3_left_torque_0 [-]"; p103 "Acceleration Trailer Brake 3 right Wheel (init) export=$sw_mec_brk_TrailerAxle3_right_angAcc$ name=mec_brk_TrailerAxle3_right_angAcc prio=1 dataSetName=std dataClassType=initIO dataClassName=initIO unit='rad/s^2' description='Acceleration Trailer Brake 3 right Wheel': interface_IO.mec_brk_TrailerAxle3_right_angAcc_0 [-]"; p104 "Angle Trailer Brake 3 right Wheel (init) export=$sw_mec_brk_TrailerAxle3_right_angPos$ name=mec_brk_TrailerAxle3_right_angPos prio=1 dataSetName=std dataClassType=initIO dataClassName=initIO unit='rad' description='Angle Trailer Brake 3 right Wheel': interface_IO.mec_brk_TrailerAxle3_right_angPos_0 [-]"; p105 "Velocity Trailer Brake 3 right Wheel (init) export=$sw_mec_brk_TrailerAxle3_right_angVel$ name=mec_brk_TrailerAxle3_right_angVel prio=1 dataSetName=std dataClassType=initIO dataClassName=initIO unit='rad/s' description='Velocity Trailer Brake 3 right Wheel': interface_IO.mec_brk_TrailerAxle3_right_angVel_0 [-]"; p106 "Torque Trailer Brake 3 right Wheel (init) export=$sw_mec_brk_TrailerAxle3_right_torque$ name=mec_brk_TrailerAxle3_right_torque prio=1 dataSetName=std dataClassType=initIO dataClassName=initIO unit='Nm' description='Torque Trailer Brake 3  right Wheel': interface_IO.mec_brk_TrailerAxle3_right_torque_0 [-]"; p107 "Torque Engine Crankshaft (init) export=$sw_mec_eng_CrankMean_torque$ name=mec_eng_CrankMean_torque prio=1 dataSetName=std dataClassType=initIO dataClassName=initIO unit='Nm' description='Torque Engine Crankshaft': interface_IO.mec_eng_CrankMean_torque_0 [-]"; p108 "Acceleration Retarder (init) export=$sw_mec_ret_Retarder_angAcc$ name=mec_ret_Retarder_angAcc prio=1 dataSetName=std dataClassType=initIO dataClassName=initIO unit='rad/s^2' description='Acceleration Retarder': interface_IO.mec_ret_Retarder_angAcc_0 [-]"; p109 "Angle Retarder (init) export=$sw_mec_ret_Retarder_angPos$ name=mec_ret_Retarder_angPos prio=1 dataSetName=std dataClassType=initIO dataClassName=initIO unit='rad' description='Angle Retarder': interface_IO.mec_ret_Retarder_angPos_0 [-]"; p110 "Velocity  Retarder (init) export=$sw_mec_ret_Retarder_angVel$ name=mec_ret_Retarder_angVel prio=1 dataSetName=std dataClassType=initIO dataClassName=initIO unit='rad/s' description='Velocity Retarder': interface_IO.mec_ret_Retarder_angVel_0 [-]"; p111 "Torque Retarder (init) export=$sw_mec_ret_Retarder_torque$ name=mec_ret_Retarder_torque prio=1 dataSetName=std dataClassType=initIO dataClassName=initIO unit='Nm' description='Torque Retarder': interface_IO.mec_ret_Retarder_torque_0 [-]"; p112 "Transmission sensor road inclination (init) export=$sw_mec_tx_inclRoadSns$ name=mec_tx_inclRoadSns prio=1 dataSetName=std dataClassType=initIO dataClassName=initIO unit='deg' description='Transmission sensor road inclination': interface_IO.mec_tx_inclRoadSns_0 [-]"; p113 "Speed sensor Transmission output (init) export=$sw_mec_tx_nGbOutD3Sns$ name=mec_tx_nGbOutD3Sns prio=1 dataSetName=std dataClassType=initIO dataClassName=initIO unit='rpm' description='Speed sensor Transmission output': interface_IO.mec_tx_nGbOutD3Sns_0 [-]"; p114 "Speed sensor Transmission output (init) export=$sw_mec_tx_nGbOutDzAwSns$ name=mec_tx_nGbOutDzAwSns prio=1 dataSetName=std dataClassType=initIO dataClassName=initIO unit='rpm' description='Speed sensor Transmission output': interface_IO.mec_tx_nGbOutDzAwSns_0 [-]"; p115 "Speed sensor Transmission output (init) export=$sw_mec_tx_nGbOutDzSfSns$ name=mec_tx_nGbOutDzSfSns prio=1 dataSetName=std dataClassType=initIO dataClassName=initIO unit='rpm' description='Speed sensor Transmission output': interface_IO.mec_tx_nGbOutDzSfSns_0 [-]"; p116 "Speed sensor Transmission output (init) export=$sw_mec_tx_nGbOutDzTuAwSns$ name=mec_tx_nGbOutDzTuAwSns prio=1 dataSetName=std dataClassType=initIO dataClassName=initIO unit='rpm' description='Speed sensor Transmission output': interface_IO.mec_tx_nGbOutDzTuAwSns_0 [-]"; p117 "Speed sensor Transmission output (init) export=$sw_mec_tx_nGbOutSns$ name=mec_tx_nGbOutSns prio=1 dataSetName=std dataClassType=initIO dataClassName=initIO unit='rpm' description='Speed sensor Transmission output': interface_IO.mec_tx_nGbOutSns_0 [-]"; p118 "Axle Load 1 (init) export=$sw_mec_veh_AxleLoad1$ name=mec_veh_AxleLoad1 prio=1 dataSetName=std dataClassType=initIO dataClassName=initIO unit='m' description='Vehicle position': interface_IO.mec_veh_AxleLoad1_0 [-]"; p119 "Axle Load 2 (init) export=$sw_mec_veh_AxleLoad2$ name=mec_veh_AxleLoad2 prio=1 dataSetName=std dataClassType=initIO dataClassName=initIO unit='m' description='Vehicle position': interface_IO.mec_veh_AxleLoad2_0 [-]"; p120 "Axle Load 3 (init) export=$sw_mec_veh_AxleLoad3$ name=mec_veh_AxleLoad3 prio=1 dataSetName=std dataClassType=initIO dataClassName=initIO unit='m' description='Vehicle position': interface_IO.mec_veh_AxleLoad3_0 [-]"; p121 "Axle Load 4 (init) export=$sw_mec_veh_AxleLoad4$ name=mec_veh_AxleLoad4 prio=1 dataSetName=std dataClassType=initIO dataClassName=initIO unit='m' description='Vehicle position': interface_IO.mec_veh_AxleLoad4_0 [-]"; p122 "Roll Coefficient Overall (init) export=$sw_mec_veh_fRollCoeffOverall$ name=mec_veh_fRollCoeffOverall prio=1 dataSetName=std dataClassType=initIO dataClassName=initIO unit='m' description='Vehicle position': interface_IO.mec_veh_fRollCoeffOverall_0 [-]"; p123 "Force Generic Vehicle Loss (init) export=$sw_mec_veh_GenericLoss_force$ name=mec_veh_GenericLoss_force prio=1 dataSetName=std dataClassType=initIO dataClassName=initIO unit='N' description='Force Generic Vehicle Loss': interface_IO.mec_veh_GenericLoss_force_0 [-]"; p124 "Acceleration Generic Vehicle Loss (init) export=$sw_mec_veh_GenericLoss_transAcc$ name=mec_veh_GenericLoss_transAcc prio=1 dataSetName=std dataClassType=initIO dataClassName=initIO unit='m/s^2' description='Acceleration Generic Vehicle Loss': interface_IO.mec_veh_GenericLoss_transAcc_0 [-]"; p125 "Position Generic Vehicle Loss (init) export=$sw_mec_veh_GenericLoss_transPos$ name=mec_veh_GenericLoss_transPos prio=1 dataSetName=std dataClassType=initIO dataClassName=initIO unit='m' description='Position Generic Vehicle Loss': interface_IO.mec_veh_GenericLoss_transPos_0 [-]"; p126 "Velocity Generic Vehicle Loss (init) export=$sw_mec_veh_GenericLoss_transVel$ name=mec_veh_GenericLoss_transVel prio=1 dataSetName=std dataClassType=initIO dataClassName=initIO unit='m/s' description='Veloctiy Generic Vehicle Loss': interface_IO.mec_veh_GenericLoss_transVel_0 [-]"; p127 "Vehicle mass (init) export=$sw_mec_veh_massVehicle$ name=mec_veh_massVehicle prio=1 dataSetName=std dataClassType=initIO dataClassName=initIO unit='kg' description='Vehicle mass': interface_IO.mec_veh_massVehicle_0 [-]"; p128 "Payload Mass (init) export=$sw_mec_veh_Payload$ name=mec_veh_Payload prio=1 dataSetName=std dataClassType=initIO dataClassName=initIO unit='m' description='Vehicle position': interface_IO.mec_veh_Payload_0 [-]"; p129 "Total GroComb Weight(init) export=$sw_mec_veh_TotalGroCombWeight$ name=mec_veh_TotalGroCombWeight prio=1 dataSetName=std dataClassType=initIO dataClassName=initIO unit='m' description='Vehicle position': interface_IO.mec_veh_TotalGroCombWeight_0 [-]"; p130 "TrailerAxle Load 1 (init) export=$sw_mec_veh_TrailerAxleLoad1$ name=mec_veh_TrailerAxleLoad1 prio=1 dataSetName=std dataClassType=initIO dataClassName=initIO unit='m' description='Vehicle position': interface_IO.mec_veh_TrailerAxleLoad1_0 [-]"; p131 "TrailerAxle Load 2 (init) export=$sw_mec_veh_TrailerAxleLoad2$ name=mec_veh_TrailerAxleLoad2 prio=1 dataSetName=std dataClassType=initIO dataClassName=initIO unit='m' description='Vehicle position': interface_IO.mec_veh_TrailerAxleLoad2_0 [-]"; p132 "TrailerAxle Load 3 (init) export=$sw_mec_veh_TrailerAxleLoad3$ name=mec_veh_TrailerAxleLoad3 prio=1 dataSetName=std dataClassType=initIO dataClassName=initIO unit='m' description='Vehicle position': interface_IO.mec_veh_TrailerAxleLoad3_0 [-]"; p133 "Vehicle acceleration (init) export=$sw_mec_veh_transAcc$ name=mec_veh_transAcc prio=1 dataSetName=std dataClassType=initIO dataClassName=initIO unit='m/s^2' description='Vehicle acceleration': interface_IO.mec_veh_transAcc_0 [-]"; p134 "Vehicle position (init) export=$sw_mec_veh_transPos$ name=mec_veh_transPos prio=1 dataSetName=std dataClassType=initIO dataClassName=initIO unit='m' description='Vehicle position': interface_IO.mec_veh_transPos_0 [-]"; p135 "Vehicle speed (real speed of vehicle) (init) export=$sw_mec_veh_transVel$ name=mec_veh_transVel prio=1 dataSetName=std dataClassType=initIO dataClassName=initIO unit='m/s' description='Vehicle speed': interface_IO.mec_veh_transVel_0 [-]"; p136 "Vehicle Speed (physical reference value) (init) export=$sw_mec_veh_VehVelReferenceCool_velocity$ name=mec_veh_VehVelReferenceCool_velocity prio=1 dataSetName=std dataClassType=initIO dataClassName=initIO unit='m/s^2' description='Vehicle Speed (physical reference value)': interface_IO.mec_veh_VehVelReferenceCool_velocity_0 [-]"; p137 "Vehicle Speed (physical reference value) (init) export=$sw_mec_veh_VehVelReferenceUhood_velocity$ name=mec_veh_VehVelReferenceUhood_velocity prio=1 dataSetName=std dataClassType=initIO dataClassName=initIO unit='m/s^2' description='Vehicle Speed (physical reference value)': interface_IO.mec_veh_VehVelReferenceUhood_velocity_0 [-]"; p138 "Acceleration Generic Wheel Loss (init) export=$sw_mec_wheel_GenericLoss_angAcc$ name=mec_wheel_GenericLoss_angAcc prio=1 dataSetName=std dataClassType=initIO dataClassName=initIO unit='rad/s^2' description='Acceleration Generic Wheel Loss': interface_IO.mec_wheel_GenericLoss_angAcc_0 [-]"; p139 "Angle Generic Wheel Loss (init) export=$sw_mec_wheel_GenericLoss_angPos$ name=mec_wheel_GenericLoss_angPos prio=1 dataSetName=std dataClassType=initIO dataClassName=initIO unit='rad' description='Angle Generic Wheel Loss': interface_IO.mec_wheel_GenericLoss_angPos_0 [-]"; p140 "Velocity Generic Wheel Loss (init) export=$sw_mec_wheel_GenericLoss_angVel$ name=mec_wheel_GenericLoss_angVel prio=1 dataSetName=std dataClassType=initIO dataClassName=initIO unit='rad/s' description='Velocity Generic Wheel Loss': interface_IO.mec_wheel_GenericLoss_angVel_0 [-]"; p141 "Torque Generic Wheel Loss (init) export=$sw_mec_wheel_GenericLoss_torque$ name=mec_wheel_GenericLoss_torque prio=1 dataSetName=std dataClassType=initIO dataClassName=initIO unit='Nm' description='Torque Generic Wheel Loss': interface_IO.mec_wheel_GenericLoss_torque_0 [-]"; p142 "[rpm] export=true prio=1 name=mec_brk_Axle1_omBrk_info dataSetName=std dataClassType=initIO dataClassName=initIO unit='rpm' description='-': mec_brk_Axle1_omBrk_info_0 [-]"; p143 "[rpm] export=true name=mec_brk_Axle1_omIn_info prio=1 dataSetName=std dataClassType=initIO dataClassName=initIO unit='rpm' description='-': mec_brk_Axle1_omIn_info_0 [-]"; p144 "[Nm] export=true prio=1 name=mec_brk_Axle1_TiBrk_info dataSetName=std dataClassType=initIO dataClassName=initIO unit='Nm' description='-': mec_brk_Axle1_TiBrk_info_0 [-]"; p145 "[Nm] export=true prio=1 name=mec_brk_Axle1_TiLoss_info dataSetName=std dataClassType=initIO dataClassName=initIO unit='Nm' description='-': mec_brk_Axle1_TiLoss_info_0 [-]"; p146 "[Nm] export=true name=mec_brk_Axle1_TIn_info prio=1 dataSetName=std dataClassType=initIO dataClassName=initIO unit='Nm' description='-': mec_brk_Axle1_TIn_info_0 [-]"; p147 "[rpm] export=true name=mec_brk_Axle2_omIn_info prio=1 dataSetName=std dataClassType=initIO dataClassName=initIO unit='rpm' description='-': mec_brk_Axle2_omIn_info_0 [-]"; p148 "[Nm] export=true prio=1 name=mec_brk_Axle2_TiBrk_info dataSetName=std dataClassType=initIO dataClassName=initIO unit='Nm' description='-': mec_brk_Axle2_TiBrk_info_0 [-]"; p149 "[Nm] export=true prio=1 name=mec_brk_Axle2_TiLoss_info dataSetName=std dataClassType=initIO dataClassName=initIO unit='Nm' description='-': mec_brk_Axle2_TiLoss_info_0 [-]"; p150 "[Nm] export=true name=mec_brk_Axle2_TIn_info prio=1 dataSetName=std dataClassType=initIO dataClassName=initIO unit='Nm' description='-': mec_brk_Axle2_TIn_info_0 [-]"; p151 "[rpm] export=true name=mec_brk_Axle3_omIn_info prio=1 dataSetName=std dataClassType=initIO dataClassName=initIO unit='rpm' description='-': mec_brk_Axle3_omIn_info_0 [-]"; p152 "[Nm] export=true prio=1 name=mec_brk_Axle3_TiBrk_info dataSetName=std dataClassType=initIO dataClassName=initIO unit='Nm' description='-': mec_brk_Axle3_TiBrk_info_0 [-]"; p153 "[Nm] export=true prio=1 name=mec_brk_Axle3_TiLoss_info dataSetName=std dataClassType=initIO dataClassName=initIO unit='Nm' description='-': mec_brk_Axle3_TiLoss_info_0 [-]"; p154 "[Nm] export=true name=mec_brk_Axle3_TIn_info prio=1 dataSetName=std dataClassType=initIO dataClassName=initIO unit='Nm' description='-': mec_brk_Axle3_TIn_info_0 [-]"; p155 "[rpm] export=true name=mec_brk_Axle4_omIn_info prio=1 dataSetName=std dataClassType=initIO dataClassName=initIO unit='rpm' description='-': mec_brk_Axle4_omIn_info_0 [-]"; p156 "[Nm] export=true prio=1 name=mec_brk_Axle4_TiBrk_info dataSetName=std dataClassType=initIO dataClassName=initIO unit='Nm' description='-': mec_brk_Axle4_TiBrk_info_0 [-]"; p157 "[Nm] export=true prio=1 name=mec_brk_Axle4_TiLoss_info dataSetName=std dataClassType=initIO dataClassName=initIO unit='Nm' description='-': mec_brk_Axle4_TiLoss_info_0 [-]"; p158 "[Nm] export=true name=mec_brk_Axle4_TIn_info prio=1 dataSetName=std dataClassType=initIO dataClassName=initIO unit='Nm' description='-': mec_brk_Axle4_TIn_info_0 [-]"; p159 "[rpm] export=true name=mec_brk_TrailerAxle1_omIn_info prio=1 dataSetName=std dataClassType=initIO dataClassName=initIO unit='rpm' description='-': mec_brk_TrailerAxle1_omIn_info_0 [-]"; p160 "[Nm] export=true prio=1 name=mec_brk_TrailerAxle1_TiBrk_info dataSetName=std dataClassType=initIO dataClassName=initIO unit='Nm' description='-': mec_brk_TrailerAxle1_TiBrk_info_0 [-]"; p161 "[Nm] export=true prio=1 name=mec_brk_TrailerAxle1_TiLoss_info dataSetName=std dataClassType=initIO dataClassName=initIO unit='Nm' description='-': mec_brk_TrailerAxle1_TiLoss_info_0 [-]"; p162 "[Nm] export=true name=mec_brk_TrailerAxle1_TIn_info prio=1 dataSetName=std dataClassType=initIO dataClassName=initIO unit='Nm' description='-': mec_brk_TrailerAxle1_TIn_info_0 [-]"; p163 "[rpm] export=true name=mec_brk_TrailerAxle2_omIn_info prio=1 dataSetName=std dataClassType=initIO dataClassName=initIO unit='rpm' description='-': mec_brk_TrailerAxle2_omIn_info_0 [-]"; p164 "[Nm] export=true prio=1 name=mec_brk_TrailerAxle2_TiBrk_info dataSetName=std dataClassType=initIO dataClassName=initIO unit='Nm' description='-': mec_brk_TrailerAxle2_TiBrk_info_0 [-]"; p165 "[Nm] export=true prio=1 name=mec_brk_TrailerAxle2_TiLoss_info dataSetName=std dataClassType=initIO dataClassName=initIO unit='Nm' description='-': mec_brk_TrailerAxle2_TiLoss_info_0 [-]"; p166 "[Nm] export=true name=mec_brk_TrailerAxle2_TIn_info prio=1 dataSetName=std dataClassType=initIO dataClassName=initIO unit='Nm' description='-': mec_brk_TrailerAxle2_TIn_info_0 [-]"; p167 "[rpm] export=true name=mec_brk_TrailerAxle3_omIn_info prio=1 dataSetName=std dataClassType=initIO dataClassName=initIO unit='rpm' description='-': mec_brk_TrailerAxle3_omIn_info_0 [-]"; p168 "[Nm] export=true prio=1 name=mec_brk_TrailerAxle3_TiBrk_info dataSetName=std dataClassType=initIO dataClassName=initIO unit='Nm' description='-': mec_brk_TrailerAxle3_TiBrk_info_0 [-]"; p169 "[Nm] export=true prio=1 name=mec_brk_TrailerAxle3_TiLoss_info dataSetName=std dataClassType=initIO dataClassName=initIO unit='Nm' description='-': mec_brk_TrailerAxle3_TiLoss_info_0 [-]"; p170 "[Nm] export=true name=mec_brk_TrailerAxle3_TIn_info prio=1 dataSetName=std dataClassType=initIO dataClassName=initIO unit='Nm' description='-': mec_brk_TrailerAxle3_TIn_info_0 [-]"; p171 "[Nm] export=true prio=1 name=mec_brk_TrailerWheel1_TiLossRollRes_info dataSetName=std dataClassType=initIO dataClassName=initIO unit='Nm' description='-': mec_brk_TrailerWheel1_TiLossRollRes_info_0 [-]"; p172 "[Nm] export=true prio=1 name=mec_brk_TrailerWheel2_TiLossRollRes_info dataSetName=std dataClassType=initIO dataClassName=initIO unit='Nm' description='-': mec_brk_TrailerWheel2_TiLossRollRes_info_0 [-]"; p173 "[Nm] export=true prio=1 name=mec_brk_TrailerWheel3_TiLossRollRes_info dataSetName=std dataClassType=initIO dataClassName=initIO unit='Nm' description='-': mec_brk_TrailerWheel3_TiLossRollRes_info_0 [-]"; p174 "[Nm] export=true prio=1 name=mec_brk_Wheel1_TiLossRollRes_info dataSetName=std dataClassType=initIO dataClassName=initIO unit='Nm' description='-': mec_brk_Wheel1_TiLossRollRes_info_0 [-]"; p175 "[Nm] export=true prio=1 name=mec_brk_Wheel2_TiLossRollRes_info dataSetName=std dataClassType=initIO dataClassName=initIO unit='Nm' description='-': mec_brk_Wheel2_TiLossRollRes_info_0 [-]"; p176 "[Nm] export=true prio=1 name=mec_brk_Wheel3_TiLossRollRes_info dataSetName=std dataClassType=initIO dataClassName=initIO unit='Nm' description='-': mec_brk_Wheel3_TiLossRollRes_info_0 [-]"; p177 "[Nm] export=true prio=1 name=mec_brk_Wheel4_TiLossRollRes_info dataSetName=std dataClassType=initIO dataClassName=initIO unit='Nm' description='-': mec_brk_Wheel4_TiLossRollRes_info_0 [-]"; p178 "[Nm] export=true name=mec_ret_T_info prio=1 dataSetName=std dataClassType=initIO dataClassName=initIO unit='Nm' description='-': mec_ret_T_info_0 [-]"; p179 "[rpm] export=true prio=1 name=mec_sht_omShtF_info dataSetName=std dataClassType=initIO dataClassName=initIO unit='rpm' description='-': mec_sht_omShtF_info_0 [-]"; p180 "[rpm] export=true prio=1 name=mec_sht_omShtR_info dataSetName=std dataClassType=initIO dataClassName=initIO unit='rpm' description='-': mec_sht_omShtR_info_0 [-]"; p181 "[rpm] export=true prio=1 name=mec_sht_TiLossShtF_info dataSetName=std dataClassType=initIO dataClassName=initIO unit='Nm' description='-': mec_sht_TiLossShtF_info_0 [-]"; p182 "[rpm] export=true prio=1 name=mec_sht_TiLossShtR_info dataSetName=std dataClassType=initIO dataClassName=initIO unit='Nm' description='-': mec_sht_TiLossShtR_info_0 [-]"; p183 "[rpm] export=true name=mec_tfc_omOut_info prio=1 dataSetName=std dataClassType=initIO dataClassName=initIO unit='rpm' description='-': mec_tfc_omOut_info_0 [-]"; p184 "[Nm] export=true prio=1 name=mec_tfc_TiLoss_info dataSetName=std dataClassType=initIO dataClassName=initIO unit='Nm' description='-': mec_tfc_TiLoss_info_0 [-]"; p185 "[Nm] export=true prio=1 name=mec_tfc_TOutFront_info dataSetName=std dataClassType=initIO dataClassName=initIO unit='Nm' description='-': mec_tfc_TOutFront_info_0 [-]"; p186 "[Nm] export=true prio=1 name=mec_tfc_TOutRear_info dataSetName=std dataClassType=initIO dataClassName=initIO unit='Nm' description='-': mec_tfc_TOutRear_info_0 [-]"; p187 "[rpm] export=true prio=1 name=mec_veh_domFW_info dataSetName=std dataClassType=initIO dataClassName=initIO unit='rpm' description='-': mec_veh_domFW_info_0 [-]"; p188 "[rad] export=true prio=1 name=mec_veh_dphiFW_info dataSetName=std dataClassType=initIO dataClassName=initIO unit='rad' description='-': mec_veh_dphiFW_info_0 [-]"; p189 "[N] export=true prio=1 name=mec_veh_FiAirDrag_info dataSetName=std dataClassType=initIO dataClassName=initIO unit='N' description='-': mec_veh_FiAirDrag_info_0 [-]"; p190 "[N] export=true prio=1 name=mec_veh_FiGradeRes_info dataSetName=std dataClassType=initIO dataClassName=initIO unit='N' description='-': mec_veh_FiGradeRes_info_0 [-]"; p191 "[N] export=true name=mec_veh_FWheelTraction_info prio=1 dataSetName=std dataClassType=initIO dataClassName=initIO unit='N' description='-': mec_veh_FWheelTraction_info_0 [-]"; p192 "[-] export=true prio=1 name=mec_veh_sFW_info dataSetName=std dataClassType=initIO dataClassName=initIO unit='-' description='-': mec_veh_sFW_info_0 [-]"; p193 "[Nm] export=true prio=1 name=mec_veh_TiFW_info dataSetName=std dataClassType=initIO dataClassName=initIO unit='Nm' description='-': mec_veh_TiFW_info_0 [-]"; p194 "[rpm] export=true prio=1 name=mec_veh_vehConfig_info dataSetName=std dataClassType=initIO dataClassName=initIO unit='rpm' description='-': mec_veh_vehConfig_info_0 [-]"; p195 "[Nm] export=true name=mec_wheel_Axle1_T_info prio=1 dataSetName=std dataClassType=initIO dataClassName=initIO unit='Nm' description='-': mec_wheel_Axle1_T_info_0 [-]"; p196 "[Nm] export=true name=mec_wheel_Axle2_T_info prio=1 dataSetName=std dataClassType=initIO dataClassName=initIO unit='Nm' description='-': mec_wheel_Axle2_T_info_0 [-]"; p197 "[Nm] export=true name=mec_wheel_Axle3_T_info prio=1 dataSetName=std dataClassType=initIO dataClassName=initIO unit='Nm' description='-': mec_wheel_Axle3_T_info_0 [-]"; p198 "[Nm] export=true name=mec_wheel_Axle4_T_info prio=1 dataSetName=std dataClassType=initIO dataClassName=initIO unit='Nm' description='-': mec_wheel_Axle4_T_info_0 [-]"; p199 "[Nm] export=true name=mec_wheel_TrailerAxle1_T_info prio=1 dataSetName=std dataClassType=initIO dataClassName=initIO unit='Nm' description='-': mec_wheel_TrailerAxle1_T_info_0 [-]"; p200 "[Nm] export=true name=mec_wheel_TrailerAxle2_T_info prio=1 dataSetName=std dataClassType=initIO dataClassName=initIO unit='Nm' description='-': mec_wheel_TrailerAxle2_T_info_0 [-]"; p201 "[Nm] export=true name=mec_wheel_TrailerAxle3_T_info prio=1 dataSetName=std dataClassType=initIO dataClassName=initIO unit='Nm' description='-': mec_wheel_TrailerAxle3_T_info_0 [-]"; p202 "Inertia propeller shaft complete [kgm^2] export=true name=JPropShaft_kgm2 prio=1 dataSetName=sht_dummy dataClassType=sht dataClassName=$dataClassNamePropShaft$ unit='kgm^2' description='Inertia Cardanshaft complete': propShaft_front.JPropShaft_kgm2 [kgm²]"; p203 "Inertia propeller shaft complete [kgm^2] export=true name=JPropShaft_kgm2 prio=1 dataSetName=sht_dummy dataClassType=sht dataClassName=$dataClassNamePropShaft$ unit='kgm^2' description='Inertia Cardanshaft complete': propShaft_rear.JPropShaft_kgm2 [kgm²]"; p204 "Ratio Retarder [-] export=true name=iRet prio=1 dataSetName=ret_dummy dataClassType=ret dataClassName=ret unit='-' description='Ratio Retarder': retarder.iRet [-]"; p205 "Inertia Retarder [kgm^2] export=true name=JRet_kgm2 prio=1 dataSetName=ret_dummy dataClassType=ret dataClassName=ret unit='kgm^2' description='Inertia Retarder': retarder.JRet_kgm2 [kgm²]"; p206 "Inertia Retarder drive Gear[kgm^2] export=true name=JRetdrvgear_kgm2 prio=1 dataSetName=ret_dummy dataClassType=ret dataClassName=ret unit='kgm^2' description='Inertia Retarder Drive Gear': retarder.JRetdrvgear_kgm2 [kgm²]"; p207 "Ratio Differential Gear [-] export=true name=iDiff prio=1 dataSetName=axle_dummy dataClassType=axle dataClassName=$dataClassNameAxle$ moduleXmlReference=$moduleXmlReferenceAxle$ unit='-' description='Ratio Differential Gear': trailerAxle1.iDiff [-]"; p208 "Is driven Axle? [-] export=true name=isDriven prio=1 dataSetName=axle_dummy dataClassType=axle dataClassName=$dataClassNameAxle$ moduleXmlReference=$moduleXmlReferenceAxle$ unit='-' description='Is Driven Axle': trailerAxle1.isDriven [-]"; p209 "Is rear Axle? [-] export=true name=isRearAxle prio=1 dataSetName=axle_dummy dataClassType=axle dataClassName=$dataClassNameAxle$ moduleXmlReference=$moduleXmlReferenceAxle$ unit='-' description='Is Rear Axle': trailerAxle1.isRearAxle [-]"; p210 "Inertia Brake Disc  [kgm^2] export=true name=JBrakeDisc_kgm2 prio=1 dataSetName=brk_dummy dataClassType=brk dataClassName=$dataClassNameBrk$ moduleXmlReference=$moduleXmlReferenceBrk$ unit='kgm^2' description='Inertia Brake Disc': trailerAxle1.JBrakeDisc_kgm2 [kgm²]"; p211 "Inertia Hub  [kgm^2] export=true name=JHub_kgm2 prio=1 dataSetName=brk_dummy dataClassType=brk dataClassName=$dataClassNameBrk$ moduleXmlReference=$moduleXmlReferenceBrk$ unit='kgm^2' description='Inertia Hub': trailerAxle1.JHub_kgm2 [-]"; p212 "Inertia Side Shaft [kgm^2] export=true name=JSideShft_kgm2 prio=1 dataSetName=axle_dummy dataClassType=axle dataClassName=$dataClassNameAxle$ moduleXmlReference=$moduleXmlReferenceAxle$ unit='kgm^2' description='Inertia Side Shaft': trailerAxle1.JSideShft_kgm2 [kgm²]"; p213 "Ratio Differential Gear [-] export=true name=iDiff prio=1 dataSetName=axle_dummy dataClassType=axle dataClassName=$dataClassNameAxle$ moduleXmlReference=$moduleXmlReferenceAxle$ unit='-' description='Ratio Differential Gear': trailerAxle2.iDiff [-]"; p214 "Is driven Axle? [-] export=true name=isDriven prio=1 dataSetName=axle_dummy dataClassType=axle dataClassName=$dataClassNameAxle$ moduleXmlReference=$moduleXmlReferenceAxle$ unit='-' description='Is Driven Axle': trailerAxle2.isDriven [-]"; p215 "Is rear Axle? [-] export=true name=isRearAxle prio=1 dataSetName=axle_dummy dataClassType=axle dataClassName=$dataClassNameAxle$ moduleXmlReference=$moduleXmlReferenceAxle$ unit='-' description='Is Rear Axle': trailerAxle2.isRearAxle [-]"; p216 "Inertia Brake Disc  [kgm^2] export=true name=JBrakeDisc_kgm2 prio=1 dataSetName=brk_dummy dataClassType=brk dataClassName=$dataClassNameBrk$ moduleXmlReference=$moduleXmlReferenceBrk$ unit='kgm^2' description='Inertia Brake Disc': trailerAxle2.JBrakeDisc_kgm2 [kgm²]"; p217 "Inertia Hub  [kgm^2] export=true name=JHub_kgm2 prio=1 dataSetName=brk_dummy dataClassType=brk dataClassName=$dataClassNameBrk$ moduleXmlReference=$moduleXmlReferenceBrk$ unit='kgm^2' description='Inertia Hub': trailerAxle2.JHub_kgm2 [-]"; p218 "Inertia Side Shaft [kgm^2] export=true name=JSideShft_kgm2 prio=1 dataSetName=axle_dummy dataClassType=axle dataClassName=$dataClassNameAxle$ moduleXmlReference=$moduleXmlReferenceAxle$ unit='kgm^2' description='Inertia Side Shaft': trailerAxle2.JSideShft_kgm2 [kgm²]"; p219 "Ratio Differential Gear [-] export=true name=iDiff prio=1 dataSetName=axle_dummy dataClassType=axle dataClassName=$dataClassNameAxle$ moduleXmlReference=$moduleXmlReferenceAxle$ unit='-' description='Ratio Differential Gear': trailerAxle3.iDiff [-]"; p220 "Is driven Axle? [-] export=true name=isDriven prio=1 dataSetName=axle_dummy dataClassType=axle dataClassName=$dataClassNameAxle$ moduleXmlReference=$moduleXmlReferenceAxle$ unit='-' description='Is Driven Axle': trailerAxle3.isDriven [-]"; p221 "Is rear Axle? [-] export=true name=isRearAxle prio=1 dataSetName=axle_dummy dataClassType=axle dataClassName=$dataClassNameAxle$ moduleXmlReference=$moduleXmlReferenceAxle$ unit='-' description='Is Rear Axle': trailerAxle3.isRearAxle [-]"; p222 "Inertia Brake Disc  [kgm^2] export=true name=JBrakeDisc_kgm2 prio=1 dataSetName=brk_dummy dataClassType=brk dataClassName=$dataClassNameBrk$ moduleXmlReference=$moduleXmlReferenceBrk$ unit='kgm^2' description='Inertia Brake Disc': trailerAxle3.JBrakeDisc_kgm2 [kgm²]"; p223 "Inertia Hub  [kgm^2] export=true name=JHub_kgm2 prio=1 dataSetName=brk_dummy dataClassType=brk dataClassName=$dataClassNameBrk$ moduleXmlReference=$moduleXmlReferenceBrk$ unit='kgm^2' description='Inertia Hub': trailerAxle3.JHub_kgm2 [-]"; p224 "Inertia Side Shaft [kgm^2] export=true name=JSideShft_kgm2 prio=1 dataSetName=axle_dummy dataClassType=axle dataClassName=$dataClassNameAxle$ moduleXmlReference=$moduleXmlReferenceAxle$ unit='kgm^2' description='Inertia Side Shaft': trailerAxle3.JSideShft_kgm2 [kgm²]"; p225 "Inertia Complete Transfer Case export=true name=JTfc_kgm2 prio=1 dataSetName=tfc_dummy dataClassType=tfc dataClassName=tfc unit='kgm^2' description='Inertia Complete Transfer Case': transferCaseA1.JTfc_kgm2 [kgm²]"; p226 "State Transfer Case export=true name=stTrfGrBoxHi prio=1 dataSetName=tfc_dummy dataClassType=tfc dataClassName=tfc unit='-' description='State Transfer Case': transferCaseA1.stTrfGrBoxHi [-]"; p227 "Air Drag Coefficient multiplied with Reference Area [m^2] export=true name=aeroCdA_m2 prio=1 dataSetName=aero_dummy dataClassType=aero dataClassName=aero unit='m^2' description='Air Drag Coefficient multiplied with Reference Area': vehicle.aeroCdA_m2 [-]"; p228 "Air Density [kg/m^3] export=true name=aeroRhoAirDensity_kgpm3 prio=1 dataSetName=aero_dummy dataClassType=aero dataClassName=aero unit='kg/m^3' description='Air Density ': vehicle.aeroRhoAirDensity_kgpm3 [-]"; p229 "number_of_weights export=true name=number_of_weights prio=1 dataSetName=massLoad_dummy dataClassType=massLoad dataClassName=massLoad unit=- description='number_of_weights': vehicle.number_of_weights [-]"; p230 "startGCW_kg export=true name=startGCW_kg prio=1 dataSetName=mass_dummy dataClassType=mass dataClassName=mass unit=kg description='startGCW_kg': vehicle.startGCW_kg [kg]"; p231 "Percentage Rolling Resistance (Rolling Resistance Coefficient) [%] export=true name=fRollCoeff prio=1 dataSetName=wheel_dummy dataClassType=wheel dataClassName=$dataClassNameWheel$ moduleXmlReference=$moduleXmlReferenceWheel$ unit='%' description='Percentage Rolling Resistance (Rolling Resistance Coefficient)': wheel_a1.fRollCoeff [-]"; p232 "Inertia Single Wheel [kgm^2] export=true name=JWheel_kgm2 prio=1 dataSetName=wheel_dummy dataClassType=wheel dataClassName=$dataClassNameWheel$ moduleXmlReference=$moduleXmlReferenceWheel$ unit='kgm^2' description='Inertia Single Wheel': wheel_a1.JWheel_kgm2 [kgm²]"; p233 "Dynamic Wheel Radius [m] export=true name=rDyn_m prio=1 dataSetName=wheel_dummy dataClassType=wheel dataClassName=$dataClassNameWheel$ moduleXmlReference=$moduleXmlReferenceWheel$ unit='m' description='Dynamic Wheel Radius': wheel_a1.rDyn_m [-]"; p234 "Percentage Rolling Resistance (Rolling Resistance Coefficient) [%] export=true name=fRollCoeff prio=1 dataSetName=wheel_dummy dataClassType=wheel dataClassName=$dataClassNameWheel$ moduleXmlReference=$moduleXmlReferenceWheel$ unit='%' description='Percentage Rolling Resistance (Rolling Resistance Coefficient)': wheel_a2.fRollCoeff [-]"; p235 "Inertia Single Wheel [kgm^2] export=true name=JWheel_kgm2 prio=1 dataSetName=wheel_dummy dataClassType=wheel dataClassName=$dataClassNameWheel$ moduleXmlReference=$moduleXmlReferenceWheel$ unit='kgm^2' description='Inertia Single Wheel': wheel_a2.JWheel_kgm2 [kgm²]"; p236 "Dynamic Wheel Radius [m] export=true name=rDyn_m prio=1 dataSetName=wheel_dummy dataClassType=wheel dataClassName=$dataClassNameWheel$ moduleXmlReference=$moduleXmlReferenceWheel$ unit='m' description='Dynamic Wheel Radius': wheel_a2.rDyn_m [-]"; p237 "Percentage Rolling Resistance (Rolling Resistance Coefficient) [%] export=true name=fRollCoeff prio=1 dataSetName=wheel_dummy dataClassType=wheel dataClassName=$dataClassNameWheel$ moduleXmlReference=$moduleXmlReferenceWheel$ unit='%' description='Percentage Rolling Resistance (Rolling Resistance Coefficient)': wheel_a3.fRollCoeff [-]"; p238 "Inertia Single Wheel [kgm^2] export=true name=JWheel_kgm2 prio=1 dataSetName=wheel_dummy dataClassType=wheel dataClassName=$dataClassNameWheel$ moduleXmlReference=$moduleXmlReferenceWheel$ unit='kgm^2' description='Inertia Single Wheel': wheel_a3.JWheel_kgm2 [kgm²]"; p239 "Dynamic Wheel Radius [m] export=true name=rDyn_m prio=1 dataSetName=wheel_dummy dataClassType=wheel dataClassName=$dataClassNameWheel$ moduleXmlReference=$moduleXmlReferenceWheel$ unit='m' description='Dynamic Wheel Radius': wheel_a3.rDyn_m [-]"; p240 "Percentage Rolling Resistance (Rolling Resistance Coefficient) [%] export=true name=fRollCoeff prio=1 dataSetName=wheel_dummy dataClassType=wheel dataClassName=$dataClassNameWheel$ moduleXmlReference=$moduleXmlReferenceWheel$ unit='%' description='Percentage Rolling Resistance (Rolling Resistance Coefficient)': wheel_a4.fRollCoeff [-]"; p241 "Inertia Single Wheel [kgm^2] export=true name=JWheel_kgm2 prio=1 dataSetName=wheel_dummy dataClassType=wheel dataClassName=$dataClassNameWheel$ moduleXmlReference=$moduleXmlReferenceWheel$ unit='kgm^2' description='Inertia Single Wheel': wheel_a4.JWheel_kgm2 [kgm²]"; p242 "Dynamic Wheel Radius [m] export=true name=rDyn_m prio=1 dataSetName=wheel_dummy dataClassType=wheel dataClassName=$dataClassNameWheel$ moduleXmlReference=$moduleXmlReferenceWheel$ unit='m' description='Dynamic Wheel Radius': wheel_a4.rDyn_m [-]"; p243 "Percentage Rolling Resistance (Rolling Resistance Coefficient) [%] export=true name=fRollCoeff prio=1 dataSetName=wheel_dummy dataClassType=wheel dataClassName=$dataClassNameWheel$ moduleXmlReference=$moduleXmlReferenceWheel$ unit='%' description='Percentage Rolling Resistance (Rolling Resistance Coefficient)': wheelTrailer_a1.fRollCoeff [-]"; p244 "Inertia Single Wheel [kgm^2] export=true name=JWheel_kgm2 prio=1 dataSetName=wheel_dummy dataClassType=wheel dataClassName=$dataClassNameWheel$ moduleXmlReference=$moduleXmlReferenceWheel$ unit='kgm^2' description='Inertia Single Wheel': wheelTrailer_a1.JWheel_kgm2 [kgm²]"; p245 "Dynamic Wheel Radius [m] export=true name=rDyn_m prio=1 dataSetName=wheel_dummy dataClassType=wheel dataClassName=$dataClassNameWheel$ moduleXmlReference=$moduleXmlReferenceWheel$ unit='m' description='Dynamic Wheel Radius': wheelTrailer_a1.rDyn_m [-]"; p246 "Percentage Rolling Resistance (Rolling Resistance Coefficient) [%] export=true name=fRollCoeff prio=1 dataSetName=wheel_dummy dataClassType=wheel dataClassName=$dataClassNameWheel$ moduleXmlReference=$moduleXmlReferenceWheel$ unit='%' description='Percentage Rolling Resistance (Rolling Resistance Coefficient)': wheelTrailer_a2.fRollCoeff [-]"; p247 "Inertia Single Wheel [kgm^2] export=true name=JWheel_kgm2 prio=1 dataSetName=wheel_dummy dataClassType=wheel dataClassName=$dataClassNameWheel$ moduleXmlReference=$moduleXmlReferenceWheel$ unit='kgm^2' description='Inertia Single Wheel': wheelTrailer_a2.JWheel_kgm2 [kgm²]"; p248 "Dynamic Wheel Radius [m] export=true name=rDyn_m prio=1 dataSetName=wheel_dummy dataClassType=wheel dataClassName=$dataClassNameWheel$ moduleXmlReference=$moduleXmlReferenceWheel$ unit='m' description='Dynamic Wheel Radius': wheelTrailer_a2.rDyn_m [-]"; p249 "Percentage Rolling Resistance (Rolling Resistance Coefficient) [%] export=true name=fRollCoeff prio=1 dataSetName=wheel_dummy dataClassType=wheel dataClassName=$dataClassNameWheel$ moduleXmlReference=$moduleXmlReferenceWheel$ unit='%' description='Percentage Rolling Resistance (Rolling Resistance Coefficient)': wheelTrailer_a3.fRollCoeff [-]"; p250 "Inertia Single Wheel [kgm^2] export=true name=JWheel_kgm2 prio=1 dataSetName=wheel_dummy dataClassType=wheel dataClassName=$dataClassNameWheel$ moduleXmlReference=$moduleXmlReferenceWheel$ unit='kgm^2' description='Inertia Single Wheel': wheelTrailer_a3.JWheel_kgm2 [kgm²]"; p251 "Dynamic Wheel Radius [m] export=true name=rDyn_m prio=1 dataSetName=wheel_dummy dataClassType=wheel dataClassName=$dataClassNameWheel$ moduleXmlReference=$moduleXmlReferenceWheel$ unit='m' description='Dynamic Wheel Radius': wheelTrailer_a3.rDyn_m [-]"; p252 "Dimension Generic Wheel Loss Torque Map export=true name=genericWheelLoss_dim prio=81 dataSetName=mecConsumers_dummy dataClassType=mecConsumers dataClassName=mecConsumers unit='' description='Dimension Generic Wheel Loss Torque Map': driveTorqueBypass1.genericWheelLoss.genericWheelLoss_dim [-]"; p253 "Dimension Generic Vehicle Loss Force Map export=true name=genericVehicleLoss_dim prio=91 dataSetName=mecConsumers_dummy dataClassType=mecConsumers dataClassName=mecConsumers unit='' description='Dimension Generic Vehicle Loss Force Map': vehicle.genericVehicleLoss.genericVehicleLoss_dim [-]"; p254 "Dimension Axle Loss Torque Map [-] export=true name=axleLoss_dim prio=1 dataSetName=axle_dummy dataClassType=axle dataClassName=$dataClassNameAxle$ moduleXmlReference=$moduleXmlReferenceAxle$ unit='-' description='Dimension Axle Loss Torque Map': axle1.axleLoss_dim [-]"; p255 "Rear Axle Loss Map [Nm] export=true name=axleLoss_map_torqueAxleIn_Nm prio=1 dataSetName=axle_dummy dataClassType=axle dataClassName=$dataClassNameAxle$ moduleXmlReference=$moduleXmlReferenceAxle$ unit='Nm' description='Rear Axle Loss Map ': axle1.axleLoss_map_torqueAxleIn_Nm [-]"; p256 "Axle Speed for Loss Torque Map [rpm] export=true name=axleLoss_x_speedAxleOut_rpm prio=1 dataSetName=axle_dummy dataClassType=axle dataClassName=$dataClassNameAxle$ moduleXmlReference=$moduleXmlReferenceAxle$ unit='rpm' description='Axle Speed for Loss Torque Map': axle1.axleLoss_x_speedAxleOut_rpm [-]"; p257 "Input Axle Torque for Loss Torque Map [Nm] export=true name=axleLoss_y_torqueAxleIn_Nm prio=1 dataSetName=axle_dummy dataClassType=axle dataClassName=$dataClassNameAxle$ moduleXmlReference=$moduleXmlReferenceAxle$ unit='Nm' description='Input Axle Torque for Loss Torque Map': axle1.axleLoss_y_torqueAxleIn_Nm [-]"; p258 "Dimension Axle Loss Torque Map [-] export=true name=axleLoss_dim prio=1 dataSetName=axle_dummy dataClassType=axle dataClassName=$dataClassNameAxle$ moduleXmlReference=$moduleXmlReferenceAxle$ unit='-' description='Dimension Axle Loss Torque Map': axle2.axleLoss_dim [-]"; p259 "Rear Axle Loss Map [Nm] export=true name=axleLoss_map_torqueAxleIn_Nm prio=1 dataSetName=axle_dummy dataClassType=axle dataClassName=$dataClassNameAxle$ moduleXmlReference=$moduleXmlReferenceAxle$ unit='Nm' description='Rear Axle Loss Map ': axle2.axleLoss_map_torqueAxleIn_Nm [-]"; p260 "Axle Speed for Loss Torque Map [rpm] export=true name=axleLoss_x_speedAxleOut_rpm prio=1 dataSetName=axle_dummy dataClassType=axle dataClassName=$dataClassNameAxle$ moduleXmlReference=$moduleXmlReferenceAxle$ unit='rpm' description='Axle Speed for Loss Torque Map': axle2.axleLoss_x_speedAxleOut_rpm [-]"; p261 "Input Axle Torque for Loss Torque Map [Nm] export=true name=axleLoss_y_torqueAxleIn_Nm prio=1 dataSetName=axle_dummy dataClassType=axle dataClassName=$dataClassNameAxle$ moduleXmlReference=$moduleXmlReferenceAxle$ unit='Nm' description='Input Axle Torque for Loss Torque Map': axle2.axleLoss_y_torqueAxleIn_Nm [-]"; p262 "Dimension Axle Loss Torque Map [-] export=true name=axleLoss_dim prio=1 dataSetName=axle_dummy dataClassType=axle dataClassName=$dataClassNameAxle$ moduleXmlReference=$moduleXmlReferenceAxle$ unit='-' description='Dimension Axle Loss Torque Map': axle3.axleLoss_dim [-]"; p263 "Rear Axle Loss Map [Nm] export=true name=axleLoss_map_torqueAxleIn_Nm prio=1 dataSetName=axle_dummy dataClassType=axle dataClassName=$dataClassNameAxle$ moduleXmlReference=$moduleXmlReferenceAxle$ unit='Nm' description='Rear Axle Loss Map ': axle3.axleLoss_map_torqueAxleIn_Nm [-]"; p264 "Axle Speed for Loss Torque Map [rpm] export=true name=axleLoss_x_speedAxleOut_rpm prio=1 dataSetName=axle_dummy dataClassType=axle dataClassName=$dataClassNameAxle$ moduleXmlReference=$moduleXmlReferenceAxle$ unit='rpm' description='Axle Speed for Loss Torque Map': axle3.axleLoss_x_speedAxleOut_rpm [-]"; p265 "Input Axle Torque for Loss Torque Map [Nm] export=true name=axleLoss_y_torqueAxleIn_Nm prio=1 dataSetName=axle_dummy dataClassType=axle dataClassName=$dataClassNameAxle$ moduleXmlReference=$moduleXmlReferenceAxle$ unit='Nm' description='Input Axle Torque for Loss Torque Map': axle3.axleLoss_y_torqueAxleIn_Nm [-]"; p266 "Dimension Axle Loss Torque Map [-] export=true name=axleLoss_dim prio=1 dataSetName=axle_dummy dataClassType=axle dataClassName=$dataClassNameAxle$ moduleXmlReference=$moduleXmlReferenceAxle$ unit='-' description='Dimension Axle Loss Torque Map': axle4.axleLoss_dim [-]"; p267 "Rear Axle Loss Map [Nm] export=true name=axleLoss_map_torqueAxleIn_Nm prio=1 dataSetName=axle_dummy dataClassType=axle dataClassName=$dataClassNameAxle$ moduleXmlReference=$moduleXmlReferenceAxle$ unit='Nm' description='Rear Axle Loss Map ': axle4.axleLoss_map_torqueAxleIn_Nm [-]"; p268 "Axle Speed for Loss Torque Map [rpm] export=true name=axleLoss_x_speedAxleOut_rpm prio=1 dataSetName=axle_dummy dataClassType=axle dataClassName=$dataClassNameAxle$ moduleXmlReference=$moduleXmlReferenceAxle$ unit='rpm' description='Axle Speed for Loss Torque Map': axle4.axleLoss_x_speedAxleOut_rpm [-]"; p269 "Input Axle Torque for Loss Torque Map [Nm] export=true name=axleLoss_y_torqueAxleIn_Nm prio=1 dataSetName=axle_dummy dataClassType=axle dataClassName=$dataClassNameAxle$ moduleXmlReference=$moduleXmlReferenceAxle$ unit='Nm' description='Input Axle Torque for Loss Torque Map': axle4.axleLoss_y_torqueAxleIn_Nm [-]"; p270 "Dimension propeller shaft Loss Torque Map  [-] export=true name=shtLoss_dim prio=1 dataSetName=sht_dummy dataClassType=sht dataClassName=$dataClassNamePropShaft$ unit='-' description='Dimension propeller shaft Loss Torque Map': propShaft_front.shtLoss_dim [-]"; p271 "Loss Torque Map Propeller Shaft [Nm] export=true name=shtLoss_map_torqueShtIn_Nm prio=1 dataSetName=sht_dummy dataClassType=sht dataClassName=$dataClassNamePropShaft$ unit='kgm^2' description='Loss Torque Map Propeller Shaft': propShaft_front.shtLoss_map_torqueShtIn_Nm [-]"; p272 "Speed Propeller Shaft for Loss Torque Map [rpm] export=true name=shtLoss_x_speedShtIn_rpm prio=1 dataSetName=sht_dummy dataClassType=sht dataClassName=$dataClassNamePropShaft$ unit='kgm^2' description='Speed Propeller Shaft for Loss Torque Map': propShaft_front.shtLoss_x_speedShtIn_rpm [-]"; p273 "Input Torque Propeller Shaft for Loss Torque Map [Nm] export=true name=shtLoss_y_torqueShtIn_Nm prio=1 dataSetName=sht_dummy dataClassType=sht dataClassName=$dataClassNamePropShaft$ unit='kgm^2' description='Input Torque Propeller Shaft for Loss Torque Map': propShaft_front.shtLoss_y_torqueShtIn_Nm [-]"; p274 "Dimension propeller shaft Loss Torque Map  [-] export=true name=shtLoss_dim prio=1 dataSetName=sht_dummy dataClassType=sht dataClassName=$dataClassNamePropShaft$ unit='-' description='Dimension propeller shaft Loss Torque Map': propShaft_rear.shtLoss_dim [-]"; p275 "Loss Torque Map Propeller Shaft [Nm] export=true name=shtLoss_map_torqueShtIn_Nm prio=1 dataSetName=sht_dummy dataClassType=sht dataClassName=$dataClassNamePropShaft$ unit='kgm^2' description='Loss Torque Map Propeller Shaft': propShaft_rear.shtLoss_map_torqueShtIn_Nm [-]"; p276 "Speed Propeller Shaft for Loss Torque Map [rpm] export=true name=shtLoss_x_speedShtIn_rpm prio=1 dataSetName=sht_dummy dataClassType=sht dataClassName=$dataClassNamePropShaft$ unit='kgm^2' description='Speed Propeller Shaft for Loss Torque Map': propShaft_rear.shtLoss_x_speedShtIn_rpm [-]"; p277 "Input Torque Propeller Shaft for Loss Torque Map [Nm] export=true name=shtLoss_y_torqueShtIn_Nm prio=1 dataSetName=sht_dummy dataClassType=sht dataClassName=$dataClassNamePropShaft$ unit='kgm^2' description='Input Torque Propeller Shaft for Loss Torque Map': propShaft_rear.shtLoss_y_torqueShtIn_Nm [-]"; p278 "Dimension Axle Loss Torque Map [-] export=true name=axleLoss_dim prio=1 dataSetName=axle_dummy dataClassType=axle dataClassName=$dataClassNameAxle$ moduleXmlReference=$moduleXmlReferenceAxle$ unit='-' description='Dimension Axle Loss Torque Map': trailerAxle1.axleLoss_dim [-]"; p279 "Rear Axle Loss Map [Nm] export=true name=axleLoss_map_torqueAxleIn_Nm prio=1 dataSetName=axle_dummy dataClassType=axle dataClassName=$dataClassNameAxle$ moduleXmlReference=$moduleXmlReferenceAxle$ unit='Nm' description='Rear Axle Loss Map ': trailerAxle1.axleLoss_map_torqueAxleIn_Nm [-]"; p280 "Axle Speed for Loss Torque Map [rpm] export=true name=axleLoss_x_speedAxleOut_rpm prio=1 dataSetName=axle_dummy dataClassType=axle dataClassName=$dataClassNameAxle$ moduleXmlReference=$moduleXmlReferenceAxle$ unit='rpm' description='Axle Speed for Loss Torque Map': trailerAxle1.axleLoss_x_speedAxleOut_rpm [-]"; p281 "Input Axle Torque for Loss Torque Map [Nm] export=true name=axleLoss_y_torqueAxleIn_Nm prio=1 dataSetName=axle_dummy dataClassType=axle dataClassName=$dataClassNameAxle$ moduleXmlReference=$moduleXmlReferenceAxle$ unit='Nm' description='Input Axle Torque for Loss Torque Map': trailerAxle1.axleLoss_y_torqueAxleIn_Nm [-]"; p282 "Dimension Axle Loss Torque Map [-] export=true name=axleLoss_dim prio=1 dataSetName=axle_dummy dataClassType=axle dataClassName=$dataClassNameAxle$ moduleXmlReference=$moduleXmlReferenceAxle$ unit='-' description='Dimension Axle Loss Torque Map': trailerAxle2.axleLoss_dim [-]"; p283 "Rear Axle Loss Map [Nm] export=true name=axleLoss_map_torqueAxleIn_Nm prio=1 dataSetName=axle_dummy dataClassType=axle dataClassName=$dataClassNameAxle$ moduleXmlReference=$moduleXmlReferenceAxle$ unit='Nm' description='Rear Axle Loss Map ': trailerAxle2.axleLoss_map_torqueAxleIn_Nm [-]"; p284 "Axle Speed for Loss Torque Map [rpm] export=true name=axleLoss_x_speedAxleOut_rpm prio=1 dataSetName=axle_dummy dataClassType=axle dataClassName=$dataClassNameAxle$ moduleXmlReference=$moduleXmlReferenceAxle$ unit='rpm' description='Axle Speed for Loss Torque Map': trailerAxle2.axleLoss_x_speedAxleOut_rpm [-]"; p285 "Input Axle Torque for Loss Torque Map [Nm] export=true name=axleLoss_y_torqueAxleIn_Nm prio=1 dataSetName=axle_dummy dataClassType=axle dataClassName=$dataClassNameAxle$ moduleXmlReference=$moduleXmlReferenceAxle$ unit='Nm' description='Input Axle Torque for Loss Torque Map': trailerAxle2.axleLoss_y_torqueAxleIn_Nm [-]"; p286 "Dimension Axle Loss Torque Map [-] export=true name=axleLoss_dim prio=1 dataSetName=axle_dummy dataClassType=axle dataClassName=$dataClassNameAxle$ moduleXmlReference=$moduleXmlReferenceAxle$ unit='-' description='Dimension Axle Loss Torque Map': trailerAxle3.axleLoss_dim [-]"; p287 "Rear Axle Loss Map [Nm] export=true name=axleLoss_map_torqueAxleIn_Nm prio=1 dataSetName=axle_dummy dataClassType=axle dataClassName=$dataClassNameAxle$ moduleXmlReference=$moduleXmlReferenceAxle$ unit='Nm' description='Rear Axle Loss Map ': trailerAxle3.axleLoss_map_torqueAxleIn_Nm [-]"; p288 "Axle Speed for Loss Torque Map [rpm] export=true name=axleLoss_x_speedAxleOut_rpm prio=1 dataSetName=axle_dummy dataClassType=axle dataClassName=$dataClassNameAxle$ moduleXmlReference=$moduleXmlReferenceAxle$ unit='rpm' description='Axle Speed for Loss Torque Map': trailerAxle3.axleLoss_x_speedAxleOut_rpm [-]"; p289 "Input Axle Torque for Loss Torque Map [Nm] export=true name=axleLoss_y_torqueAxleIn_Nm prio=1 dataSetName=axle_dummy dataClassType=axle dataClassName=$dataClassNameAxle$ moduleXmlReference=$moduleXmlReferenceAxle$ unit='Nm' description='Input Axle Torque for Loss Torque Map': trailerAxle3.axleLoss_y_torqueAxleIn_Nm [-]"; p290 "Gear Ratio Transfer Case export=true name=iTfc prio=1 dataSetName=tfc_dummy dataClassType=tfc dataClassName=tfc unit='-' description='Gear Ratio Transfer Case': transferCaseA1.iTfc [-]"; p291 "Dimension Loss Torque Map Transfer Case export=true name=tfcLoss_dim prio=1 dataSetName=tfc_dummy dataClassType=tfc dataClassName=tfc unit='-' description='Dimension Loss Torque Map Transfer Case': transferCaseA1.tfcLoss_dim [-]"; p292 "Loss Torque Map Transfer Case export=true name=tfcLoss_map_torqueTfcIn_Nm prio=1 dataSetName=tfc_dummy dataClassType=tfc dataClassName=tfc unit='Nm' description='Loss Torque Map Transfer Case': transferCaseA1.tfcLoss_map_torqueTfcIn_Nm [Nm]"; p293 "Input Speed for Loss Torque Map Transfer Case export=true name=tfcLoss_x_speedTfcIn_rpm prio=1 dataSetName=tfc_dummy dataClassType=tfc dataClassName=tfc unit='rpm' description='Output Speed for Loss Torque Map Transfer Case': transferCaseA1.tfcLoss_x_speedTfcIn_rpm [-]"; p294 "Input Torque for Loss Torque Map Transfer Case export=true name=tfcLoss_y_torqueTfcIn_Nm prio=1 dataSetName=tfc_dummy dataClassType=tfc dataClassName=tfc unit='Nm' description='Input Torque for Loss Torque Map Transfer Case': transferCaseA1.tfcLoss_y_torqueTfcIn_Nm [-]"; p295 "Torque Distribution Transfer Case export=true name=torqueDistribution prio=1 dataSetName=tfc_dummy dataClassType=tfc dataClassName=tfc unit='-' description='Torque Distribution Transfer Case': transferCaseA1.torqueDistribution [-]"; p296 "mass_distribution export=true name=mass_distribution prio=1 dataSetName=massLoad_dummy dataClassType=massLoad dataClassName=massLoad unit=- description='Mass Distribution': vehicle.mass_distribution [-]"; p297 "Air Compressor Speed for Loss Torque Map [rpm] export=true name=genericWheelLoss_x_speed_rpm prio=82 dataSetName=mecConsumers_dummy dataClassType=mecConsumers dataClassName=mecConsumers unit='rpm' description='Generic Wheel Speed for Loss Torque Map [rpm]': driveTorqueBypass1.genericWheelLoss.genericWheelLoss_x_speed_rpm [-]"; p298 "Generic Wheel Loss Torque Map [Nm] export=true name=genericWheelLoss_map_lossTorque_Nm prio=83 dataSetName=mecConsumers_dummy dataClassType=mecConsumers dataClassName=mecConsumers unit='Nm' description='Generic Wheel Loss Torque Map [Nm]': driveTorqueBypass1.genericWheelLoss.genericWheelLoss_map_lossTorque_Nm [Nm]"; p299 "Generic Vehicle Speed for Loss Force Map [rpm] export=true name=genericVehicleLoss_x_velocity_kmh prio=92 dataSetName=mecConsumers_dummy dataClassType=mecConsumers dataClassName=mecConsumers unit='rpm' description='Generic Vehicle Speed for Loss Force Map [rpm]': vehicle.genericVehicleLoss.genericVehicleLoss_x_velocity_kmh [-]"; p300 "Generic Vehicle Loss Force Map [Nm] export=true name=genericVehicleLoss_map_loss_N prio=93 dataSetName=mecConsumers_dummy dataClassType=mecConsumers dataClassName=mecConsumers unit='Nm' description='Generic Vehicle Loss Force Map [Nm]': vehicle.genericVehicleLoss.genericVehicleLoss_map_loss_N [Nm]"
      mask help: Generated by SimulationX 4.2.2.68604
      mask init:
      | if ~isempty(initCmd), try, evalin('base', initCmd); end, end
      mask Display: disp('mec_pointmass_generic_ATvoith_std_sf'); port_label('input', 1, 'cpc_cdA_offset'); port_label('input', 2, 'env_curv_pm'); port_label('input', 3, 'env_density'); port_label('input', 4, 'env_load_massdiff'); port_label('input', 5, 'env_road_slope_pct'); port_label('input', 6, 'mec_brk_Axle1_left_torque'); port_label('input', 7, 'mec_brk_Axle1_right_torque'); port_label('input', 8, 'mec_brk_Axle2_left_torque'); port_label('input', 9, 'mec_brk_Axle2_right_torque'); port_label('input', 10, 'mec_brk_Axle3_left_torque'); port_label('input', 11, 'mec_brk_Axle3_right_torque'); port_label('input', 12, 'mec_brk_Axle4_left_torque'); port_label('input', 13, 'mec_brk_Axle4_right_torque'); port_label('input', 14, 'mec_brk_TrailerAxle1_left_torque'); port_label('input', 15, 'mec_brk_TrailerAxle1_right_torque'); port_label('input', 16, 'mec_brk_TrailerAxle2_left_torque'); port_label('input', 17, 'mec_brk_TrailerAxle2_right_torque'); port_label('input', 18, 'mec_brk_TrailerAxle3_left_torque'); port_label('input', 19, 'mec_brk_TrailerAxle3_right_torque'); port_label('input', 20, 'mec_eng_CrankMean_torque'); port_label('input', 21, 'mec_ret_Retarder_torque'); port_label('input', 22, 'mec_veh_GenericLoss_force'); port_label('input', 23, 'mec_wheel_GenericLoss_torque'); port_label('output', 1, 'mec_brk_Axle1_angAcc'); port_label('output', 2, 'mec_brk_Axle1_angPos'); port_label('output', 3, 'mec_brk_Axle1_angVel'); port_label('output', 4, 'mec_brk_Axle2_angAcc'); port_label('output', 5, 'mec_brk_Axle2_angPos'); port_label('output', 6, 'mec_brk_Axle2_angVel'); port_label('output', 7, 'mec_brk_Axle3_angAcc'); port_label('output', 8, 'mec_brk_Axle3_angPos'); port_label('output', 9, 'mec_brk_Axle3_angVel'); port_label('output', 10, 'mec_brk_Axle4_angAcc'); port_label('output', 11, 'mec_brk_Axle4_angPos'); port_label('output', 12, 'mec_brk_Axle4_angVel'); port_label('output', 13, 'mec_brk_TrailerAxle1_angAcc'); port_label('output', 14, 'mec_brk_TrailerAxle1_angPos'); port_label('output', 15, 'mec_brk_TrailerAxle1_angVel'); port_label('output', 16, 'mec_brk_TrailerAxle2_angAcc'); port_label('output', 17, 'mec_brk_TrailerAxle2_angPos'); port_label('output', 18, 'mec_brk_TrailerAxle2_angVel'); port_label('output', 19, 'mec_brk_TrailerAxle3_angAcc'); port_label('output', 20, 'mec_brk_TrailerAxle3_angPos'); port_label('output', 21, 'mec_brk_TrailerAxle3_angVel'); port_label('output', 22, 'mec_brk_Axle1_omBrk_info'); port_label('output', 23, 'mec_brk_Axle1_omIn_info'); port_label('output', 24, 'mec_brk_Axle1_TiBrk_info'); port_label('output', 25, 'mec_brk_Axle1_TiLoss_info'); port_label('output', 26, 'mec_brk_Axle1_TIn_info'); port_label('output', 27, 'mec_brk_Axle2_omIn_info'); port_label('output', 28, 'mec_brk_Axle2_TiBrk_info'); port_label('output', 29, 'mec_brk_Axle2_TiLoss_info'); port_label('output', 30, 'mec_brk_Axle2_TIn_info'); port_label('output', 31, 'mec_brk_Axle3_omIn_info'); port_label('output', 32, 'mec_brk_Axle3_TiBrk_info'); port_label('output', 33, 'mec_brk_Axle3_TiLoss_info'); port_label('output', 34, 'mec_brk_Axle3_TIn_info'); port_label('output', 35, 'mec_brk_Axle4_omIn_info'); port_label('output', 36, 'mec_brk_Axle4_TiBrk_info'); port_label('output', 37, 'mec_brk_Axle4_TiLoss_info'); port_label('output', 38, 'mec_brk_Axle4_TIn_info'); port_label('output', 39, 'mec_brk_TrailerAxle1_omIn_info'); port_label('output', 40, 'mec_brk_TrailerAxle1_TiBrk_info'); port_label('output', 41, 'mec_brk_TrailerAxle1_TiLoss_info'); port_label('output', 42, 'mec_brk_TrailerAxle1_TIn_info'); port_label('output', 43, 'mec_brk_TrailerAxle2_omIn_info'); port_label('output', 44, 'mec_brk_TrailerAxle2_TiBrk_info'); port_label('output', 45, 'mec_brk_TrailerAxle2_TiLoss_info'); port_label('output', 46, 'mec_brk_TrailerAxle2_TIn_info'); port_label('output', 47, 'mec_brk_TrailerAxle3_omIn_info'); port_label('output', 48, 'mec_brk_TrailerAxle3_TiBrk_info'); port_label('output', 49, 'mec_brk_TrailerAxle3_TiLoss_info'); port_label('output', 50, 'mec_brk_TrailerAxle3_TIn_info'); port_label('output', 51, 'mec_brk_TrailerWheel1_TiLossRollRes_info'); port_label('output', 52, 'mec_brk_TrailerWheel2_TiLossRollRes_info'); port_label('output', 53, 'mec_brk_TrailerWheel3_TiLossRollRes_info'); port_label('output', 54, 'mec_brk_Wheel1_TiLossRollRes_info'); port_label('output', 55, 'mec_brk_Wheel2_TiLossRollRes_info'); port_label('output', 56, 'mec_brk_Wheel3_TiLossRollRes_info'); port_label('output', 57, 'mec_brk_Wheel4_TiLossRollRes_info'); port_label('output', 58, 'mec_ret_T_info'); port_label('output', 59, 'mec_sht_omShtF_info'); port_label('output', 60, 'mec_sht_omShtR_info'); port_label('output', 61, 'mec_sht_TiLossShtF_info'); port_label('output', 62, 'mec_sht_TiLossShtR_info'); port_label('output', 63, 'mec_tfc_omOut_info'); port_label('output', 64, 'mec_tfc_TiLoss_info'); port_label('output', 65, 'mec_tfc_TOutFront_info'); port_label('output', 66, 'mec_tfc_TOutRear_info'); port_label('output', 67, 'mec_veh_domFW_info'); port_label('output', 68, 'mec_veh_dphiFW_info'); port_label('output', 69, 'mec_veh_FiAirDrag_info'); port_label('output', 70, 'mec_veh_FiGradeRes_info'); port_label('output', 71, 'mec_veh_FWheelTraction_info'); port_label('output', 72, 'mec_veh_sFW_info'); port_label('output', 73, 'mec_veh_TiFW_info'); port_label('output', 74, 'mec_veh_vehConfig_info'); port_label('output', 75, 'mec_wheel_Axle1_T_info'); port_label('output', 76, 'mec_wheel_Axle2_T_info'); port_label('output', 77, 'mec_wheel_Axle3_T_info'); port_label('output', 78, 'mec_wheel_Axle4_T_info'); port_label('output', 79, 'mec_wheel_TrailerAxle1_T_info'); port_label('output', 80, 'mec_wheel_TrailerAxle2_T_info'); port_label('output', 81, 'mec_wheel_TrailerAxle3_T_info'); port_label('output', 82, 'mec_brk_Axle1_left_angAcc'); port_label('output', 83, 'mec_brk_Axle1_left_angPos'); port_label('output', 84, 'mec_brk_Axle1_left_angVel'); port_label('output', 85, 'mec_brk_Axle1_right_angAcc'); port_label('output', 86, 'mec_brk_Axle1_right_angPos'); port_label('output', 87, 'mec_brk_Axle1_right_angVel'); port_label('output', 88, 'mec_brk_Axle2_left_angAcc'); port_label('output', 89, 'mec_brk_Axle2_left_angPos'); port_label('output', 90, 'mec_brk_Axle2_left_angVel'); port_label('output', 91, 'mec_brk_Axle2_right_angAcc'); port_label('output', 92, 'mec_brk_Axle2_right_angPos'); port_label('output', 93, 'mec_brk_Axle2_right_angVel'); port_label('output', 94, 'mec_brk_Axle3_left_angAcc'); port_label('output', 95, 'mec_brk_Axle3_left_angPos'); port_label('output', 96, 'mec_brk_Axle3_left_angVel'); port_label('output', 97, 'mec_brk_Axle3_right_angAcc'); port_label('output', 98, 'mec_brk_Axle3_right_angPos'); port_label('output', 99, 'mec_brk_Axle3_right_angVel'); port_label('output', 100, 'mec_brk_Axle4_left_angAcc'); port_label('output', 101, 'mec_brk_Axle4_left_angPos'); port_label('output', 102, 'mec_brk_Axle4_left_angVel'); port_label('output', 103, 'mec_brk_Axle4_right_angAcc'); port_label('output', 104, 'mec_brk_Axle4_right_angPos'); port_label('output', 105, 'mec_brk_Axle4_right_angVel'); port_label('output', 106, 'mec_brk_TrailerAxle1_left_angAcc'); port_label('output', 107, 'mec_brk_TrailerAxle1_left_angPos'); port_label('output', 108, 'mec_brk_TrailerAxle1_left_angVel'); port_label('output', 109, 'mec_brk_TrailerAxle1_right_angAcc'); port_label('output', 110, 'mec_brk_TrailerAxle1_right_angPos'); port_label('output', 111, 'mec_brk_TrailerAxle1_right_angVel'); port_label('output', 112, 'mec_brk_TrailerAxle2_left_angAcc'); port_label('output', 113, 'mec_brk_TrailerAxle2_left_angPos'); port_label('output', 114, 'mec_brk_TrailerAxle2_left_angVel'); port_label('output', 115, 'mec_brk_TrailerAxle2_right_angAcc'); port_label('output', 116, 'mec_brk_TrailerAxle2_right_angPos'); port_label('output', 117, 'mec_brk_TrailerAxle2_right_angVel'); port_label('output', 118, 'mec_brk_TrailerAxle3_left_angAcc'); port_label('output', 119, 'mec_brk_TrailerAxle3_left_angPos'); port_label('output', 120, 'mec_brk_TrailerAxle3_left_angVel'); port_label('output', 121, 'mec_brk_TrailerAxle3_right_angAcc'); port_label('output', 122, 'mec_brk_TrailerAxle3_right_angPos'); port_label('output', 123, 'mec_brk_TrailerAxle3_right_angVel'); port_label('output', 124, 'mec_ret_Retarder_angAcc'); port_label('output', 125, 'mec_ret_Retarder_angPos'); port_label('output', 126, 'mec_ret_Retarder_angVel'); port_label('output', 127, 'mec_veh_GenericLoss_transAcc'); port_label('output', 128, 'mec_veh_GenericLoss_transPos'); port_label('output', 129, 'mec_veh_GenericLoss_transVel'); port_label('output', 130, 'mec_veh_VehVelReferenceCool_velocity'); port_label('output', 131, 'mec_veh_VehVelReferenceUhood_velocity'); port_label('output', 132, 'mec_wheel_GenericLoss_angAcc'); port_label('output', 133, 'mec_wheel_GenericLoss_angPos'); port_label('output', 134, 'mec_wheel_GenericLoss_angVel'); port_label('output', 135, 'mec_tx_inclRoadSns'); port_label('output', 136, 'mec_tx_nGbOutD3Sns'); port_label('output', 137, 'mec_tx_nGbOutDzAwSns'); port_label('output', 138, 'mec_tx_nGbOutDzSfSns'); port_label('output', 139, 'mec_tx_nGbOutDzTuAwSns'); port_label('output', 140, 'mec_tx_nGbOutSns'); port_label('output', 141, 'mec_veh_AxleLoad1'); port_label('output', 142, 'mec_veh_AxleLoad2'); port_label('output', 143, 'mec_veh_AxleLoad3'); port_label('output', 144, 'mec_veh_AxleLoad4'); port_label('output', 145, 'mec_veh_fRollCoeffOverall'); port_label('output', 146, 'mec_veh_massVehicle'); port_label('output', 147, 'mec_veh_Payload'); port_label('output', 148, 'mec_veh_TotalGroCombWeight'); port_label('output', 149, 'mec_veh_TrailerAxleLoad1'); port_label('output', 150, 'mec_veh_TrailerAxleLoad2'); port_label('output', 151, 'mec_veh_TrailerAxleLoad3'); port_label('output', 152, 'mec_veh_transAcc'); port_label('output', 153, 'mec_veh_transPos'); port_label('output', 154, 'mec_veh_transVel');
  mec_brk_Axle1_angAcc : Outport
  mec_brk_Axle1_angPos : Outport  Port=2
  mec_brk_Axle1_angVel : Outport  Port=3
  mec_brk_Axle2_angAcc : Outport  Port=4
  mec_brk_Axle2_angPos : Outport  Port=5
  mec_brk_Axle2_angVel : Outport  Port=6
  mec_brk_Axle3_angAcc : Outport  Port=7
  mec_brk_Axle3_angPos : Outport  Port=8
  mec_brk_Axle3_angVel : Outport  Port=9
  mec_brk_Axle4_angAcc : Outport  Port=10
  mec_brk_Axle4_angPos : Outport  Port=11
  mec_brk_Axle4_angVel : Outport  Port=12
  mec_brk_TrailerAxle1_angAcc : Outport  Port=13
  mec_brk_TrailerAxle1_angPos : Outport  Port=14
  mec_brk_TrailerAxle1_angVel : Outport  Port=15
  mec_brk_TrailerAxle2_angAcc : Outport  Port=16
  mec_brk_TrailerAxle2_angPos : Outport  Port=17
  mec_brk_TrailerAxle2_angVel : Outport  Port=18
  mec_brk_TrailerAxle3_angAcc : Outport  Port=19
  mec_brk_TrailerAxle3_angPos : Outport  Port=20
  mec_brk_TrailerAxle3_angVel : Outport  Port=21
  mec_brk_Axle1_omBrk_info : Outport  Port=22
  mec_brk_Axle1_omIn_info : Outport  Port=23
  mec_brk_Axle1_TiBrk_info : Outport  Port=24
  mec_brk_Axle1_TiLoss_info : Outport  Port=25
  mec_brk_Axle1_TIn_info : Outport  Port=26
  mec_brk_Axle2_omIn_info : Outport  Port=27
  mec_brk_Axle2_TiBrk_info : Outport  Port=28
  mec_brk_Axle2_TiLoss_info : Outport  Port=29
  mec_brk_Axle2_TIn_info : Outport  Port=30
  mec_brk_Axle3_omIn_info : Outport  Port=31
  mec_brk_Axle3_TiBrk_info : Outport  Port=32
  mec_brk_Axle3_TiLoss_info : Outport  Port=33
  mec_brk_Axle3_TIn_info : Outport  Port=34
  mec_brk_Axle4_omIn_info : Outport  Port=35
  mec_brk_Axle4_TiBrk_info : Outport  Port=36
  mec_brk_Axle4_TiLoss_info : Outport  Port=37
  mec_brk_Axle4_TIn_info : Outport  Port=38
  mec_brk_TrailerAxle1_omIn_info : Outport  Port=39
  mec_brk_TrailerAxle1_TiBrk_info : Outport  Port=40
  mec_brk_TrailerAxle1_TiLoss_info : Outport  Port=41
  mec_brk_TrailerAxle1_TIn_info : Outport  Port=42
  mec_brk_TrailerAxle2_omIn_info : Outport  Port=43
  mec_brk_TrailerAxle2_TiBrk_info : Outport  Port=44
  mec_brk_TrailerAxle2_TiLoss_info : Outport  Port=45
  mec_brk_TrailerAxle2_TIn_info : Outport  Port=46
  mec_brk_TrailerAxle3_omIn_info : Outport  Port=47
  mec_brk_TrailerAxle3_TiBrk_info : Outport  Port=48
  mec_brk_TrailerAxle3_TiLoss_info : Outport  Port=49
  mec_brk_TrailerAxle3_TIn_info : Outport  Port=50
  mec_brk_TrailerWheel1_TiLossRollRes_info : Outport  Port=51
  mec_brk_TrailerWheel2_TiLossRollRes_info : Outport  Port=52
  mec_brk_TrailerWheel3_TiLossRollRes_info : Outport  Port=53
  mec_brk_Wheel1_TiLossRollRes_info : Outport  Port=54
  mec_brk_Wheel2_TiLossRollRes_info : Outport  Port=55
  mec_brk_Wheel3_TiLossRollRes_info : Outport  Port=56
  mec_brk_Wheel4_TiLossRollRes_info : Outport  Port=57
  mec_ret_T_info : Outport  Port=58
  mec_sht_omShtF_info : Outport  Port=59
  mec_sht_omShtR_info : Outport  Port=60
  mec_sht_TiLossShtF_info : Outport  Port=61
  mec_sht_TiLossShtR_info : Outport  Port=62
  mec_tfc_omOut_info : Outport  Port=63
  mec_tfc_TiLoss_info : Outport  Port=64
  mec_tfc_TOutFront_info : Outport  Port=65
  mec_tfc_TOutRear_info : Outport  Port=66
  mec_veh_domFW_info : Outport  Port=67
  mec_veh_dphiFW_info : Outport  Port=68
  mec_veh_FiAirDrag_info : Outport  Port=69
  mec_veh_FiGradeRes_info : Outport  Port=70
  mec_veh_FWheelTraction_info : Outport  Port=71
  mec_veh_sFW_info : Outport  Port=72
  mec_veh_TiFW_info : Outport  Port=73
  mec_veh_vehConfig_info : Outport  Port=74
  mec_wheel_Axle1_T_info : Outport  Port=75
  mec_wheel_Axle2_T_info : Outport  Port=76
  mec_wheel_Axle3_T_info : Outport  Port=77
  mec_wheel_Axle4_T_info : Outport  Port=78
  mec_wheel_TrailerAxle1_T_info : Outport  Port=79
  mec_wheel_TrailerAxle2_T_info : Outport  Port=80
  mec_wheel_TrailerAxle3_T_info : Outport  Port=81
  mec_brk_Axle1_left_angAcc : Outport  Port=82
  mec_brk_Axle1_left_angPos : Outport  Port=83
  mec_brk_Axle1_left_angVel : Outport  Port=84
  mec_brk_Axle1_right_angAcc : Outport  Port=85
  mec_brk_Axle1_right_angPos : Outport  Port=86
  mec_brk_Axle1_right_angVel : Outport  Port=87
  mec_brk_Axle2_left_angAcc : Outport  Port=88
  mec_brk_Axle2_left_angPos : Outport  Port=89
  mec_brk_Axle2_left_angVel : Outport  Port=90
  mec_brk_Axle2_right_angAcc : Outport  Port=91
  mec_brk_Axle2_right_angPos : Outport  Port=92
  mec_brk_Axle2_right_angVel : Outport  Port=93
  mec_brk_Axle3_left_angAcc : Outport  Port=94
  mec_brk_Axle3_left_angPos : Outport  Port=95
  mec_brk_Axle3_left_angVel : Outport  Port=96
  mec_brk_Axle3_right_angAcc : Outport  Port=97
  mec_brk_Axle3_right_angPos : Outport  Port=98
  mec_brk_Axle3_right_angVel : Outport  Port=99
  mec_brk_Axle4_left_angAcc : Outport  Port=100
  mec_brk_Axle4_left_angPos : Outport  Port=101
  mec_brk_Axle4_left_angVel : Outport  Port=102
  mec_brk_Axle4_right_angAcc : Outport  Port=103
  mec_brk_Axle4_right_angPos : Outport  Port=104
  mec_brk_Axle4_right_angVel : Outport  Port=105
  mec_brk_TrailerAxle1_left_angAcc : Outport  Port=106
  mec_brk_TrailerAxle1_left_angPos : Outport  Port=107
  mec_brk_TrailerAxle1_left_angVel : Outport  Port=108
  mec_brk_TrailerAxle1_right_angAcc : Outport  Port=109
  mec_brk_TrailerAxle1_right_angPos : Outport  Port=110
  mec_brk_TrailerAxle1_right_angVel : Outport  Port=111
  mec_brk_TrailerAxle2_left_angAcc : Outport  Port=112
  mec_brk_TrailerAxle2_left_angPos : Outport  Port=113
  mec_brk_TrailerAxle2_left_angVel : Outport  Port=114
  mec_brk_TrailerAxle2_right_angAcc : Outport  Port=115
  mec_brk_TrailerAxle2_right_angPos : Outport  Port=116
  mec_brk_TrailerAxle2_right_angVel : Outport  Port=117
  mec_brk_TrailerAxle3_left_angAcc : Outport  Port=118
  mec_brk_TrailerAxle3_left_angPos : Outport  Port=119
  mec_brk_TrailerAxle3_left_angVel : Outport  Port=120
  mec_brk_TrailerAxle3_right_angAcc : Outport  Port=121
  mec_brk_TrailerAxle3_right_angPos : Outport  Port=122
  mec_brk_TrailerAxle3_right_angVel : Outport  Port=123
  mec_ret_Retarder_angAcc : Outport  Port=124
  mec_ret_Retarder_angPos : Outport  Port=125
  mec_ret_Retarder_angVel : Outport  Port=126
  mec_veh_GenericLoss_transAcc : Outport  Port=127
  mec_veh_GenericLoss_transPos : Outport  Port=128
  mec_veh_GenericLoss_transVel : Outport  Port=129
  mec_veh_VehVelReferenceCool_velocity : Outport  Port=130
  mec_veh_VehVelReferenceUhood_velocity : Outport  Port=131
  mec_wheel_GenericLoss_angAcc : Outport  Port=132
  mec_wheel_GenericLoss_angPos : Outport  Port=133
  mec_wheel_GenericLoss_angVel : Outport  Port=134
  mec_tx_inclRoadSns : Outport  Port=135
  mec_tx_nGbOutD3Sns : Outport  Port=136
  mec_tx_nGbOutDzAwSns : Outport  Port=137
  mec_tx_nGbOutDzSfSns : Outport  Port=138
  mec_tx_nGbOutDzTuAwSns : Outport  Port=139
  mec_tx_nGbOutSns : Outport  Port=140
  mec_veh_AxleLoad1 : Outport  Port=141
  mec_veh_AxleLoad2 : Outport  Port=142
  mec_veh_AxleLoad3 : Outport  Port=143
  mec_veh_AxleLoad4 : Outport  Port=144
  mec_veh_fRollCoeffOverall : Outport  Port=145
  mec_veh_massVehicle : Outport  Port=146
  mec_veh_Payload : Outport  Port=147
  mec_veh_TotalGroCombWeight : Outport  Port=148
  mec_veh_TrailerAxleLoad1 : Outport  Port=149
  mec_veh_TrailerAxleLoad2 : Outport  Port=150
  mec_veh_TrailerAxleLoad3 : Outport  Port=151
  mec_veh_transAcc : Outport  Port=152
  mec_veh_transPos : Outport  Port=153
  mec_veh_transVel : Outport  Port=154
  wires:
  mec_pointmass_generic_ATvoith_std_sf/154 -> mec_veh_transVel/1  "mec_veh_transVel"
  mec_pointmass_generic_ATvoith_std_sf/153 -> mec_veh_transPos/1  "mec_veh_transPos"
  mec_pointmass_generic_ATvoith_std_sf/152 -> mec_veh_transAcc/1  "mec_veh_transAcc"
  mec_pointmass_generic_ATvoith_std_sf/151 -> mec_veh_TrailerAxleLoad3/1  "mec_veh_TrailerAxleLoad3"
  mec_pointmass_generic_ATvoith_std_sf/150 -> mec_veh_TrailerAxleLoad2/1  "mec_veh_TrailerAxleLoad2"
  mec_pointmass_generic_ATvoith_std_sf/149 -> mec_veh_TrailerAxleLoad1/1  "mec_veh_TrailerAxleLoad1"
  mec_pointmass_generic_ATvoith_std_sf/148 -> mec_veh_TotalGroCombWeight/1  "mec_veh_TotalGroCombWeight"
  mec_pointmass_generic_ATvoith_std_sf/147 -> mec_veh_Payload/1  "mec_veh_Payload"
  mec_pointmass_generic_ATvoith_std_sf/146 -> mec_veh_massVehicle/1  "mec_veh_massVehicle"
  mec_pointmass_generic_ATvoith_std_sf/145 -> mec_veh_fRollCoeffOverall/1  "mec_veh_fRollCoeffOverall"
  mec_pointmass_generic_ATvoith_std_sf/144 -> mec_veh_AxleLoad4/1  "mec_veh_AxleLoad4"
  mec_pointmass_generic_ATvoith_std_sf/143 -> mec_veh_AxleLoad3/1  "mec_veh_AxleLoad3"
  mec_pointmass_generic_ATvoith_std_sf/142 -> mec_veh_AxleLoad2/1  "mec_veh_AxleLoad2"
  mec_pointmass_generic_ATvoith_std_sf/141 -> mec_veh_AxleLoad1/1  "mec_veh_AxleLoad1"
  mec_pointmass_generic_ATvoith_std_sf/140 -> mec_tx_nGbOutSns/1  "mec_tx_nGbOutSns"
  mec_pointmass_generic_ATvoith_std_sf/139 -> mec_tx_nGbOutDzTuAwSns/1  "mec_tx_nGbOutDzTuAwSns"
  mec_pointmass_generic_ATvoith_std_sf/138 -> mec_tx_nGbOutDzSfSns/1  "mec_tx_nGbOutDzSfSns"
  mec_pointmass_generic_ATvoith_std_sf/137 -> mec_tx_nGbOutDzAwSns/1  "mec_tx_nGbOutDzAwSns"
  mec_pointmass_generic_ATvoith_std_sf/136 -> mec_tx_nGbOutD3Sns/1  "mec_tx_nGbOutD3Sns"
  mec_pointmass_generic_ATvoith_std_sf/135 -> mec_tx_inclRoadSns/1  "mec_tx_inclRoadSns"
  mec_pointmass_generic_ATvoith_std_sf/134 -> mec_wheel_GenericLoss_angVel/1  "mec_wheel_GenericLoss_angVel"
  mec_pointmass_generic_ATvoith_std_sf/133 -> mec_wheel_GenericLoss_angPos/1  "mec_wheel_GenericLoss_angPos"
  mec_pointmass_generic_ATvoith_std_sf/132 -> mec_wheel_GenericLoss_angAcc/1  "mec_wheel_GenericLoss_angAcc"
  mec_pointmass_generic_ATvoith_std_sf/131 -> mec_veh_VehVelReferenceUhood_velocity/1  "mec_veh_VehVelReferenceUhood_velocity"
  mec_pointmass_generic_ATvoith_std_sf/130 -> mec_veh_VehVelReferenceCool_velocity/1  "mec_veh_VehVelReferenceCool_velocity"
  mec_pointmass_generic_ATvoith_std_sf/129 -> mec_veh_GenericLoss_transVel/1  "mec_veh_GenericLoss_transVel"
  mec_pointmass_generic_ATvoith_std_sf/128 -> mec_veh_GenericLoss_transPos/1  "mec_veh_GenericLoss_transPos"
  mec_pointmass_generic_ATvoith_std_sf/127 -> mec_veh_GenericLoss_transAcc/1  "mec_veh_GenericLoss_transAcc"
  mec_pointmass_generic_ATvoith_std_sf/126 -> mec_ret_Retarder_angVel/1  "mec_ret_Retarder_angVel"
  mec_pointmass_generic_ATvoith_std_sf/125 -> mec_ret_Retarder_angPos/1  "mec_ret_Retarder_angPos"
  mec_pointmass_generic_ATvoith_std_sf/124 -> mec_ret_Retarder_angAcc/1  "mec_ret_Retarder_angAcc"
  mec_pointmass_generic_ATvoith_std_sf/123 -> mec_brk_TrailerAxle3_right_angVel/1  "mec_brk_TrailerAxle3_right_angVel"
  mec_pointmass_generic_ATvoith_std_sf/122 -> mec_brk_TrailerAxle3_right_angPos/1  "mec_brk_TrailerAxle3_right_angPos"
  mec_pointmass_generic_ATvoith_std_sf/121 -> mec_brk_TrailerAxle3_right_angAcc/1  "mec_brk_TrailerAxle3_right_angAcc"
  mec_pointmass_generic_ATvoith_std_sf/120 -> mec_brk_TrailerAxle3_left_angVel/1  "mec_brk_TrailerAxle3_left_angVel"
  mec_pointmass_generic_ATvoith_std_sf/119 -> mec_brk_TrailerAxle3_left_angPos/1  "mec_brk_TrailerAxle3_left_angPos"
  mec_pointmass_generic_ATvoith_std_sf/118 -> mec_brk_TrailerAxle3_left_angAcc/1  "mec_brk_TrailerAxle3_left_angAcc"
  mec_pointmass_generic_ATvoith_std_sf/117 -> mec_brk_TrailerAxle2_right_angVel/1  "mec_brk_TrailerAxle2_right_angVel"
  mec_pointmass_generic_ATvoith_std_sf/116 -> mec_brk_TrailerAxle2_right_angPos/1  "mec_brk_TrailerAxle2_right_angPos"
  mec_pointmass_generic_ATvoith_std_sf/115 -> mec_brk_TrailerAxle2_right_angAcc/1  "mec_brk_TrailerAxle2_right_angAcc"
  mec_pointmass_generic_ATvoith_std_sf/114 -> mec_brk_TrailerAxle2_left_angVel/1  "mec_brk_TrailerAxle2_left_angVel"
  mec_pointmass_generic_ATvoith_std_sf/113 -> mec_brk_TrailerAxle2_left_angPos/1  "mec_brk_TrailerAxle2_left_angPos"
  mec_pointmass_generic_ATvoith_std_sf/112 -> mec_brk_TrailerAxle2_left_angAcc/1  "mec_brk_TrailerAxle2_left_angAcc"
  mec_pointmass_generic_ATvoith_std_sf/111 -> mec_brk_TrailerAxle1_right_angVel/1  "mec_brk_TrailerAxle1_right_angVel"
  mec_pointmass_generic_ATvoith_std_sf/110 -> mec_brk_TrailerAxle1_right_angPos/1  "mec_brk_TrailerAxle1_right_angPos"
  mec_pointmass_generic_ATvoith_std_sf/109 -> mec_brk_TrailerAxle1_right_angAcc/1  "mec_brk_TrailerAxle1_right_angAcc"
  mec_pointmass_generic_ATvoith_std_sf/108 -> mec_brk_TrailerAxle1_left_angVel/1  "mec_brk_TrailerAxle1_left_angVel"
  mec_pointmass_generic_ATvoith_std_sf/107 -> mec_brk_TrailerAxle1_left_angPos/1  "mec_brk_TrailerAxle1_left_angPos"
  mec_pointmass_generic_ATvoith_std_sf/106 -> mec_brk_TrailerAxle1_left_angAcc/1  "mec_brk_TrailerAxle1_left_angAcc"
  mec_pointmass_generic_ATvoith_std_sf/105 -> mec_brk_Axle4_right_angVel/1  "mec_brk_Axle4_right_angVel"
  mec_pointmass_generic_ATvoith_std_sf/104 -> mec_brk_Axle4_right_angPos/1  "mec_brk_Axle4_right_angPos"
  mec_pointmass_generic_ATvoith_std_sf/103 -> mec_brk_Axle4_right_angAcc/1  "mec_brk_Axle4_right_angAcc"
  mec_pointmass_generic_ATvoith_std_sf/102 -> mec_brk_Axle4_left_angVel/1  "mec_brk_Axle4_left_angVel"
  mec_pointmass_generic_ATvoith_std_sf/101 -> mec_brk_Axle4_left_angPos/1  "mec_brk_Axle4_left_angPos"
  mec_pointmass_generic_ATvoith_std_sf/100 -> mec_brk_Axle4_left_angAcc/1  "mec_brk_Axle4_left_angAcc"
  mec_pointmass_generic_ATvoith_std_sf/99 -> mec_brk_Axle3_right_angVel/1  "mec_brk_Axle3_right_angVel"
  mec_pointmass_generic_ATvoith_std_sf/98 -> mec_brk_Axle3_right_angPos/1  "mec_brk_Axle3_right_angPos"
  mec_pointmass_generic_ATvoith_std_sf/97 -> mec_brk_Axle3_right_angAcc/1  "mec_brk_Axle3_right_angAcc"
  mec_pointmass_generic_ATvoith_std_sf/96 -> mec_brk_Axle3_left_angVel/1  "mec_brk_Axle3_left_angVel"
  mec_pointmass_generic_ATvoith_std_sf/95 -> mec_brk_Axle3_left_angPos/1  "mec_brk_Axle3_left_angPos"
  mec_pointmass_generic_ATvoith_std_sf/94 -> mec_brk_Axle3_left_angAcc/1  "mec_brk_Axle3_left_angAcc"
  mec_pointmass_generic_ATvoith_std_sf/93 -> mec_brk_Axle2_right_angVel/1  "mec_brk_Axle2_right_angVel"
  mec_pointmass_generic_ATvoith_std_sf/92 -> mec_brk_Axle2_right_angPos/1  "mec_brk_Axle2_right_angPos"
  mec_pointmass_generic_ATvoith_std_sf/91 -> mec_brk_Axle2_right_angAcc/1  "mec_brk_Axle2_right_angAcc"
  mec_pointmass_generic_ATvoith_std_sf/90 -> mec_brk_Axle2_left_angVel/1  "mec_brk_Axle2_left_angVel"
  mec_pointmass_generic_ATvoith_std_sf/89 -> mec_brk_Axle2_left_angPos/1  "mec_brk_Axle2_left_angPos"
  mec_pointmass_generic_ATvoith_std_sf/88 -> mec_brk_Axle2_left_angAcc/1  "mec_brk_Axle2_left_angAcc"
  mec_pointmass_generic_ATvoith_std_sf/87 -> mec_brk_Axle1_right_angVel/1  "mec_brk_Axle1_right_angVel"
  mec_pointmass_generic_ATvoith_std_sf/86 -> mec_brk_Axle1_right_angPos/1  "mec_brk_Axle1_right_angPos"
  mec_pointmass_generic_ATvoith_std_sf/85 -> mec_brk_Axle1_right_angAcc/1  "mec_brk_Axle1_right_angAcc"
  mec_pointmass_generic_ATvoith_std_sf/84 -> mec_brk_Axle1_left_angVel/1  "mec_brk_Axle1_left_angVel"
  mec_pointmass_generic_ATvoith_std_sf/83 -> mec_brk_Axle1_left_angPos/1  "mec_brk_Axle1_left_angPos"
  mec_pointmass_generic_ATvoith_std_sf/82 -> mec_brk_Axle1_left_angAcc/1  "mec_brk_Axle1_left_angAcc"
  mec_pointmass_generic_ATvoith_std_sf/81 -> mec_wheel_TrailerAxle3_T_info/1  "mec_wheel_TrailerAxle3_T_info"
  mec_pointmass_generic_ATvoith_std_sf/80 -> mec_wheel_TrailerAxle2_T_info/1  "mec_wheel_TrailerAxle2_T_info"
  mec_pointmass_generic_ATvoith_std_sf/79 -> mec_wheel_TrailerAxle1_T_info/1  "mec_wheel_TrailerAxle1_T_info"
  mec_pointmass_generic_ATvoith_std_sf/78 -> mec_wheel_Axle4_T_info/1  "mec_wheel_Axle4_T_info"
  mec_pointmass_generic_ATvoith_std_sf/77 -> mec_wheel_Axle3_T_info/1  "mec_wheel_Axle3_T_info"
  mec_pointmass_generic_ATvoith_std_sf/76 -> mec_wheel_Axle2_T_info/1  "mec_wheel_Axle2_T_info"
  mec_pointmass_generic_ATvoith_std_sf/75 -> mec_wheel_Axle1_T_info/1  "mec_wheel_Axle1_T_info"
  mec_pointmass_generic_ATvoith_std_sf/74 -> mec_veh_vehConfig_info/1  "mec_veh_vehConfig_info"
  mec_pointmass_generic_ATvoith_std_sf/73 -> mec_veh_TiFW_info/1  "mec_veh_TiFW_info"
  mec_pointmass_generic_ATvoith_std_sf/72 -> mec_veh_sFW_info/1  "mec_veh_sFW_info"
  mec_pointmass_generic_ATvoith_std_sf/71 -> mec_veh_FWheelTraction_info/1  "mec_veh_FWheelTraction_info"
  mec_pointmass_generic_ATvoith_std_sf/70 -> mec_veh_FiGradeRes_info/1  "mec_veh_FiGradeRes_info"
  mec_pointmass_generic_ATvoith_std_sf/69 -> mec_veh_FiAirDrag_info/1  "mec_veh_FiAirDrag_info"
  mec_pointmass_generic_ATvoith_std_sf/68 -> mec_veh_dphiFW_info/1  "mec_veh_dphiFW_info"
  mec_pointmass_generic_ATvoith_std_sf/67 -> mec_veh_domFW_info/1  "mec_veh_domFW_info"
  mec_pointmass_generic_ATvoith_std_sf/66 -> mec_tfc_TOutRear_info/1  "mec_tfc_TOutRear_info"
  mec_pointmass_generic_ATvoith_std_sf/65 -> mec_tfc_TOutFront_info/1  "mec_tfc_TOutFront_info"
  mec_pointmass_generic_ATvoith_std_sf/64 -> mec_tfc_TiLoss_info/1  "mec_tfc_TiLoss_info"
  mec_pointmass_generic_ATvoith_std_sf/63 -> mec_tfc_omOut_info/1  "mec_tfc_omOut_info"
  mec_pointmass_generic_ATvoith_std_sf/62 -> mec_sht_TiLossShtR_info/1  "mec_sht_TiLossShtR_info"
  mec_pointmass_generic_ATvoith_std_sf/61 -> mec_sht_TiLossShtF_info/1  "mec_sht_TiLossShtF_info"
  mec_pointmass_generic_ATvoith_std_sf/60 -> mec_sht_omShtR_info/1  "mec_sht_omShtR_info"
  mec_pointmass_generic_ATvoith_std_sf/59 -> mec_sht_omShtF_info/1  "mec_sht_omShtF_info"
  mec_pointmass_generic_ATvoith_std_sf/58 -> mec_ret_T_info/1  "mec_ret_T_info"
  mec_pointmass_generic_ATvoith_std_sf/57 -> mec_brk_Wheel4_TiLossRollRes_info/1  "mec_brk_Wheel4_TiLossRollRes_info"
  mec_pointmass_generic_ATvoith_std_sf/56 -> mec_brk_Wheel3_TiLossRollRes_info/1  "mec_brk_Wheel3_TiLossRollRes_info"
  mec_pointmass_generic_ATvoith_std_sf/55 -> mec_brk_Wheel2_TiLossRollRes_info/1  "mec_brk_Wheel2_TiLossRollRes_info"
  mec_pointmass_generic_ATvoith_std_sf/54 -> mec_brk_Wheel1_TiLossRollRes_info/1  "mec_brk_Wheel1_TiLossRollRes_info"
  mec_pointmass_generic_ATvoith_std_sf/53 -> mec_brk_TrailerWheel3_TiLossRollRes_info/1  "mec_brk_TrailerWheel3_TiLossRollRes_info"
  mec_pointmass_generic_ATvoith_std_sf/52 -> mec_brk_TrailerWheel2_TiLossRollRes_info/1  "mec_brk_TrailerWheel2_TiLossRollRes_info"
  mec_pointmass_generic_ATvoith_std_sf/51 -> mec_brk_TrailerWheel1_TiLossRollRes_info/1  "mec_brk_TrailerWheel1_TiLossRollRes_info"
  mec_pointmass_generic_ATvoith_std_sf/50 -> mec_brk_TrailerAxle3_TIn_info/1  "mec_brk_TrailerAxle3_TIn_info"
  mec_pointmass_generic_ATvoith_std_sf/49 -> mec_brk_TrailerAxle3_TiLoss_info/1  "mec_brk_TrailerAxle3_TiLoss_info"
  mec_pointmass_generic_ATvoith_std_sf/48 -> mec_brk_TrailerAxle3_TiBrk_info/1  "mec_brk_TrailerAxle3_TiBrk_info"
  mec_pointmass_generic_ATvoith_std_sf/47 -> mec_brk_TrailerAxle3_omIn_info/1  "mec_brk_TrailerAxle3_omIn_info"
  mec_pointmass_generic_ATvoith_std_sf/46 -> mec_brk_TrailerAxle2_TIn_info/1  "mec_brk_TrailerAxle2_TIn_info"
  mec_pointmass_generic_ATvoith_std_sf/45 -> mec_brk_TrailerAxle2_TiLoss_info/1  "mec_brk_TrailerAxle2_TiLoss_info"
  mec_pointmass_generic_ATvoith_std_sf/44 -> mec_brk_TrailerAxle2_TiBrk_info/1  "mec_brk_TrailerAxle2_TiBrk_info"
  mec_pointmass_generic_ATvoith_std_sf/43 -> mec_brk_TrailerAxle2_omIn_info/1  "mec_brk_TrailerAxle2_omIn_info"
  mec_pointmass_generic_ATvoith_std_sf/42 -> mec_brk_TrailerAxle1_TIn_info/1  "mec_brk_TrailerAxle1_TIn_info"
  mec_pointmass_generic_ATvoith_std_sf/41 -> mec_brk_TrailerAxle1_TiLoss_info/1  "mec_brk_TrailerAxle1_TiLoss_info"
  mec_pointmass_generic_ATvoith_std_sf/40 -> mec_brk_TrailerAxle1_TiBrk_info/1  "mec_brk_TrailerAxle1_TiBrk_info"
  mec_pointmass_generic_ATvoith_std_sf/39 -> mec_brk_TrailerAxle1_omIn_info/1  "mec_brk_TrailerAxle1_omIn_info"
  mec_pointmass_generic_ATvoith_std_sf/38 -> mec_brk_Axle4_TIn_info/1  "mec_brk_Axle4_TIn_info"
  mec_pointmass_generic_ATvoith_std_sf/37 -> mec_brk_Axle4_TiLoss_info/1  "mec_brk_Axle4_TiLoss_info"
  mec_pointmass_generic_ATvoith_std_sf/36 -> mec_brk_Axle4_TiBrk_info/1  "mec_brk_Axle4_TiBrk_info"
  mec_pointmass_generic_ATvoith_std_sf/35 -> mec_brk_Axle4_omIn_info/1  "mec_brk_Axle4_omIn_info"
  mec_pointmass_generic_ATvoith_std_sf/34 -> mec_brk_Axle3_TIn_info/1  "mec_brk_Axle3_TIn_info"
  mec_pointmass_generic_ATvoith_std_sf/33 -> mec_brk_Axle3_TiLoss_info/1  "mec_brk_Axle3_TiLoss_info"
  mec_pointmass_generic_ATvoith_std_sf/32 -> mec_brk_Axle3_TiBrk_info/1  "mec_brk_Axle3_TiBrk_info"
  mec_pointmass_generic_ATvoith_std_sf/31 -> mec_brk_Axle3_omIn_info/1  "mec_brk_Axle3_omIn_info"
  mec_pointmass_generic_ATvoith_std_sf/30 -> mec_brk_Axle2_TIn_info/1  "mec_brk_Axle2_TIn_info"
  mec_pointmass_generic_ATvoith_std_sf/29 -> mec_brk_Axle2_TiLoss_info/1  "mec_brk_Axle2_TiLoss_info"
  mec_pointmass_generic_ATvoith_std_sf/28 -> mec_brk_Axle2_TiBrk_info/1  "mec_brk_Axle2_TiBrk_info"
  mec_pointmass_generic_ATvoith_std_sf/27 -> mec_brk_Axle2_omIn_info/1  "mec_brk_Axle2_omIn_info"
  mec_pointmass_generic_ATvoith_std_sf/26 -> mec_brk_Axle1_TIn_info/1  "mec_brk_Axle1_TIn_info"
  mec_pointmass_generic_ATvoith_std_sf/25 -> mec_brk_Axle1_TiLoss_info/1  "mec_brk_Axle1_TiLoss_info"
  mec_pointmass_generic_ATvoith_std_sf/24 -> mec_brk_Axle1_TiBrk_info/1  "mec_brk_Axle1_TiBrk_info"
  mec_pointmass_generic_ATvoith_std_sf/23 -> mec_brk_Axle1_omIn_info/1  "mec_brk_Axle1_omIn_info"
  mec_pointmass_generic_ATvoith_std_sf/22 -> mec_brk_Axle1_omBrk_info/1  "mec_brk_Axle1_omBrk_info"
  mec_pointmass_generic_ATvoith_std_sf/21 -> mec_brk_TrailerAxle3_angVel/1  "mec_brk_TrailerAxle3_angVel"
  mec_pointmass_generic_ATvoith_std_sf/20 -> mec_brk_TrailerAxle3_angPos/1  "mec_brk_TrailerAxle3_angPos"
  mec_pointmass_generic_ATvoith_std_sf/19 -> mec_brk_TrailerAxle3_angAcc/1  "mec_brk_TrailerAxle3_angAcc"
  mec_pointmass_generic_ATvoith_std_sf/18 -> mec_brk_TrailerAxle2_angVel/1  "mec_brk_TrailerAxle2_angVel"
  mec_pointmass_generic_ATvoith_std_sf/17 -> mec_brk_TrailerAxle2_angPos/1  "mec_brk_TrailerAxle2_angPos"
  mec_pointmass_generic_ATvoith_std_sf/16 -> mec_brk_TrailerAxle2_angAcc/1  "mec_brk_TrailerAxle2_angAcc"
  mec_pointmass_generic_ATvoith_std_sf/15 -> mec_brk_TrailerAxle1_angVel/1  "mec_brk_TrailerAxle1_angVel"
  mec_pointmass_generic_ATvoith_std_sf/14 -> mec_brk_TrailerAxle1_angPos/1  "mec_brk_TrailerAxle1_angPos"
  mec_pointmass_generic_ATvoith_std_sf/13 -> mec_brk_TrailerAxle1_angAcc/1  "mec_brk_TrailerAxle1_angAcc"
  mec_pointmass_generic_ATvoith_std_sf/12 -> mec_brk_Axle4_angVel/1  "mec_brk_Axle4_angVel"
  mec_pointmass_generic_ATvoith_std_sf/11 -> mec_brk_Axle4_angPos/1  "mec_brk_Axle4_angPos"
  mec_pointmass_generic_ATvoith_std_sf/10 -> mec_brk_Axle4_angAcc/1  "mec_brk_Axle4_angAcc"
  mec_pointmass_generic_ATvoith_std_sf/9 -> mec_brk_Axle3_angVel/1  "mec_brk_Axle3_angVel"
  mec_pointmass_generic_ATvoith_std_sf/8 -> mec_brk_Axle3_angPos/1  "mec_brk_Axle3_angPos"
  mec_pointmass_generic_ATvoith_std_sf/7 -> mec_brk_Axle3_angAcc/1  "mec_brk_Axle3_angAcc"
  mec_pointmass_generic_ATvoith_std_sf/6 -> mec_brk_Axle2_angVel/1  "mec_brk_Axle2_angVel"
  mec_pointmass_generic_ATvoith_std_sf/5 -> mec_brk_Axle2_angPos/1  "mec_brk_Axle2_angPos"
  mec_pointmass_generic_ATvoith_std_sf/4 -> mec_brk_Axle2_angAcc/1  "mec_brk_Axle2_angAcc"
  mec_pointmass_generic_ATvoith_std_sf/3 -> mec_brk_Axle1_angVel/1  "mec_brk_Axle1_angVel"
  mec_pointmass_generic_ATvoith_std_sf/2 -> mec_brk_Axle1_angPos/1  "mec_brk_Axle1_angPos"
  mec_pointmass_generic_ATvoith_std_sf/1 -> mec_brk_Axle1_angAcc/1  "mec_brk_Axle1_angAcc"
  mec_wheel_GenericLoss_torque/1 -> mec_pointmass_generic_ATvoith_std_sf/23  "mec_wheel_GenericLoss_torque"
  mec_veh_GenericLoss_force/1 -> mec_pointmass_generic_ATvoith_std_sf/22  "mec_veh_GenericLoss_force"
  mec_ret_Retarder_torque/1 -> mec_pointmass_generic_ATvoith_std_sf/21  "mec_ret_Retarder_torque"
  mec_eng_CrankMean_torque/1 -> mec_pointmass_generic_ATvoith_std_sf/20  "mec_eng_CrankMean_torque"
  mec_brk_TrailerAxle3_right_torque/1 -> mec_pointmass_generic_ATvoith_std_sf/19  "mec_brk_TrailerAxle3_right_torque"
  mec_brk_TrailerAxle3_left_torque/1 -> mec_pointmass_generic_ATvoith_std_sf/18  "mec_brk_TrailerAxle3_left_torque"
  mec_brk_TrailerAxle2_right_torque/1 -> mec_pointmass_generic_ATvoith_std_sf/17  "mec_brk_TrailerAxle2_right_torque"
  mec_brk_TrailerAxle2_left_torque/1 -> mec_pointmass_generic_ATvoith_std_sf/16  "mec_brk_TrailerAxle2_left_torque"
  mec_brk_TrailerAxle1_right_torque/1 -> mec_pointmass_generic_ATvoith_std_sf/15  "mec_brk_TrailerAxle1_right_torque"
  mec_brk_TrailerAxle1_left_torque/1 -> mec_pointmass_generic_ATvoith_std_sf/14  "mec_brk_TrailerAxle1_left_torque"
  mec_brk_Axle4_right_torque/1 -> mec_pointmass_generic_ATvoith_std_sf/13  "mec_brk_Axle4_right_torque"
  mec_brk_Axle4_left_torque/1 -> mec_pointmass_generic_ATvoith_std_sf/12  "mec_brk_Axle4_left_torque"
  mec_brk_Axle3_right_torque/1 -> mec_pointmass_generic_ATvoith_std_sf/11  "mec_brk_Axle3_right_torque"
  mec_brk_Axle3_left_torque/1 -> mec_pointmass_generic_ATvoith_std_sf/10  "mec_brk_Axle3_left_torque"
  mec_brk_Axle2_right_torque/1 -> mec_pointmass_generic_ATvoith_std_sf/9  "mec_brk_Axle2_right_torque"
  mec_brk_Axle2_left_torque/1 -> mec_pointmass_generic_ATvoith_std_sf/8  "mec_brk_Axle2_left_torque"
  mec_brk_Axle1_right_torque/1 -> mec_pointmass_generic_ATvoith_std_sf/7  "mec_brk_Axle1_right_torque"
  mec_brk_Axle1_left_torque/1 -> mec_pointmass_generic_ATvoith_std_sf/6  "mec_brk_Axle1_left_torque"
  env_road_slope_pct/1 -> mec_pointmass_generic_ATvoith_std_sf/5  "env_road_slope_pct"
  env_load_massdiff/1 -> mec_pointmass_generic_ATvoith_std_sf/4  "env_load_massdiff"
  env_density/1 -> mec_pointmass_generic_ATvoith_std_sf/3  "env_density"
  env_curv_pm/1 -> mec_pointmass_generic_ATvoith_std_sf/2  "env_curv_pm"
  cpc_cdA_offset/1 -> mec_pointmass_generic_ATvoith_std_sf/1  "cpc_cdA_offset"
